simulink model "sim_tcyb_2024_pos_ctrl"  (R2020a)
settings: Solver=ode4  StartTime=0.0  StopTime=30.0  FixedStep=0.01  RelTol=1e-3
values from neighbouring files (symbols this model uses):
  alfa_theta = 20    [init_tcyb_2024_pos_ctrl.m]
  alfa_theta_obs = 100    [init_tcyb_2024_pos_ctrl.m]
  c1_diff_sigma_bar_v = diag([25; 30; 20])    [init_tcyb_2024_pos_ctrl.m]
  c1v = diag([5.8; 6.5; 6.5])    [init_tcyb_2024_pos_ctrl.m]
  c2_diff_sigma_bar_v = diag([50; 50; 10])    [init_tcyb_2024_pos_ctrl.m]
  c2v = diag([5.8; 6.5; 6.5])    [init_tcyb_2024_pos_ctrl.m]
  c3_diff_sigma_bar_v = diag([15; 15; 10])    [init_tcyb_2024_pos_ctrl.m]
  c3v = diag([4.8; 6.4; 6.0])    [init_tcyb_2024_pos_ctrl.m]
  c_psi_p = [0.05; 0.05; 0.05]    [init_tcyb_2024_pos_ctrl.m]
  delta_p_i_0 = zeros(3, NF)    [init_tcyb_2024_pos_ctrl.m]
  delta_v_i_0 = zeros(3, NF)    [init_tcyb_2024_pos_ctrl.m]
  dp_aa_t = 0.2 * ones(3, 5) + ( 1.0 - 0.2 ) * rand(3, 5)    [init_tcyb_2024_pos_ctrl.m]
  dp_ff_t = [ 0.4 * ones(1, 5) + ( 1.0 - 0.4 ) * rand(1, 5);                      0.4 * ones(1, 5) + ( 1.0 - 0.4 ) * rand(1, 5);                      0.2 * ones(1, 5) + ( 0.6 - 0.2 ) * rand(1, 5) ]    [init_tcyb_2024_pos_ctrl.m]
  dp_phi_t = ( - pi / 2 ) * ones(3, 5) + ( pi / 2 - ( - pi / 2 ) ) * rand(3, 5)    [init_tcyb_2024_pos_ctrl.m]
  etai_0 = zeros(3,5)    [init_tcyb_2024_pos_ctrl.m]
  kai_1_t = 0.02    [init_tcyb_2024_pos_ctrl.m]
  kai_3_t = 0.1    [init_tcyb_2024_pos_ctrl.m]
  ksii_0 = zeros(3,5)    [init_tcyb_2024_pos_ctrl.m]
  l1v = diag([20; 20; 20])    [init_tcyb_2024_pos_ctrl.m]
  l2v = diag([30; 30; 30])    [init_tcyb_2024_pos_ctrl.m]
  Lamd_diff_sigma_bar_v = 0.5    [init_tcyb_2024_pos_ctrl.m]
  mass_i = zeros(1,NF)    [init_tcyb_2024_pos_ctrl.m]
  Mii = diag([1;0;0;0;1])    [init_tcyb_2024_pos_ctrl.m]
  pos0 = zeros(3, 1)    [init_tcyb_2024_pos_ctrl.m]
  PZ0 = P0(3)    [init_tcyb_2024_pos_ctrl.m]
  PZ1 = 10    [init_tcyb_2024_pos_ctrl.m]
  Qci_init = repmat([1;0;0;0],1,NF)    [init_tcyb_2024_pos_ctrl.m]
  R0 = 4    [init_tcyb_2024_pos_ctrl.m]
  R1 = 8    [init_tcyb_2024_pos_ctrl.m]
  rho_p = [0.1; 0.1; 0.1]    [init_tcyb_2024_pos_ctrl.m]
  Rx2 = 10    [init_tcyb_2024_pos_ctrl.m]
  Ry2 = 6    [init_tcyb_2024_pos_ctrl.m]
  Rz2 = 4    [init_tcyb_2024_pos_ctrl.m]
  T0 = 0    [init_tcyb_2024_pos_ctrl.m]
  T1 = tseq1    (= 10)    [init_tcyb_2024_pos_ctrl.m]
  T12 = tseq1 + tseq12    (= 20)    [init_tcyb_2024_pos_ctrl.m]
  T2 = tseq1 + tseq12 + tseq2    (= 30)    [init_tcyb_2024_pos_ctrl.m]
  tau_p = 5    [init_tcyb_2024_pos_ctrl.m]
  theta0 = ( 2 / 5 ) * pi    (= 1.25663706144)    [init_tcyb_2024_pos_ctrl.m]
  vel0 = zeros(3, 1)    [init_tcyb_2024_pos_ctrl.m]
  Wij = [0,0,1,0,0;              0,0,1,1,0;              1,0,0,0,1;              0,1,1,0,0;              0,0,1,0,0]    [init_tcyb_2024_pos_ctrl.m]
  X1 = 8    [init_tcyb_2024_pos_ctrl.m]
  X2 = 2    [init_tcyb_2024_pos_ctrl.m]
  X3 = 3    [init_tcyb_2024_pos_ctrl.m]
  Y1 = 10    [init_tcyb_2024_pos_ctrl.m]
  Y2 = 2    [init_tcyb_2024_pos_ctrl.m]
  Y3 = 4    [init_tcyb_2024_pos_ctrl.m]
  Z1 = 4    [init_tcyb_2024_pos_ctrl.m]
  Z2 = -6    [init_tcyb_2024_pos_ctrl.m]
  Z3 = 2    [init_tcyb_2024_pos_ctrl.m]
  zeta_diff_sigma_bar_v = 0.08    [init_tcyb_2024_pos_ctrl.m]
undefined symbols (not defined in the file or in its folder): cal_frac_squ, p_alfav1, p_alfav2, p_gamma1_pos, p_gamma1_vel, p_gamma2_pos, p_gamma2_vel, q_alfav1, q_alfav2, q_gamma1_pos, q_gamma1_vel, q_gamma2_pos, q_gamma2_vel
(part 1 of 4)
settings Model: Creator=zzy  LastModifiedBy=Hershey.A
settings DataIOCC: ReturnWorkspaceOutputs=off
settings DebuggingCC: ArithmeticOperatorsInVariantConditions=warning
settings SFSimCC: SimUseLocalCustomCode=off  CustomCodeUndefinedFunction=UseInterfaceOnly
settings RTWCC: RTWUseLocalCustomCode=off

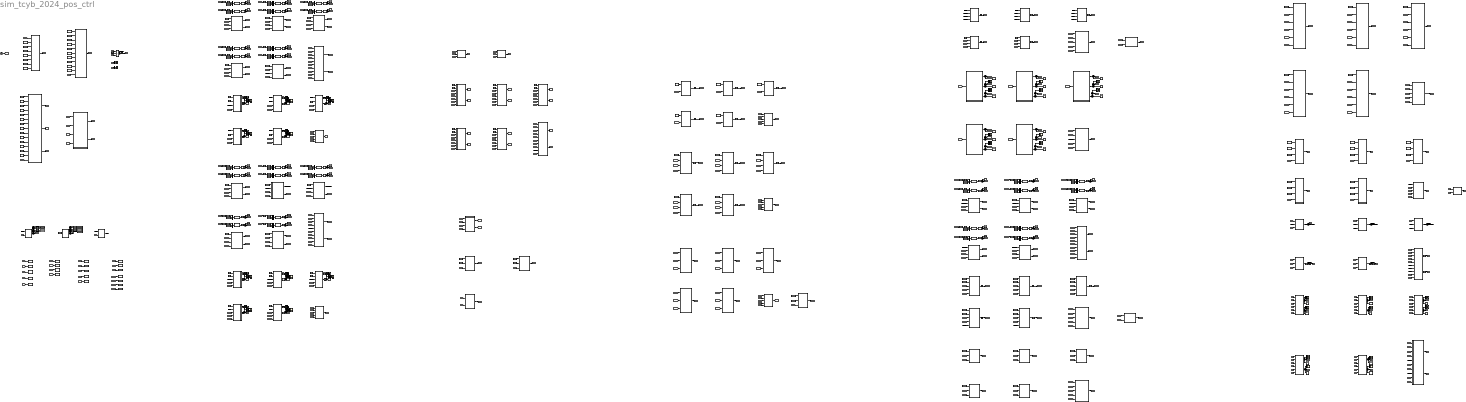
== system sim_tcyb_2024_pos_ctrl ==
  Add{,1..9} (10 alike) : Sum
  Clock : Clock
  Constant : Constant  Value=T1
  Constant{1,4,15,224,228,233,237,242} (8 alike) : Constant  Value=Mii
  Constant{10..14} (5 alike) : Constant  Value=tau_p
  Constant{100,102,107,112,117} (5 alike) : Constant  Value=p_alfav1
  Constant{101,103,108,113,118} (5 alike) : Constant  Value=alfa_theta
  Constant{97,104,109,114,119} (5 alike) : Constant  Value=q_alfav1
  Constant{98,105,110,115,120} (5 alike) : Constant  Value=p_alfav2
  Constant{99,106,111,116,121} (5 alike) : Constant  Value=q_alfav2
  Constant{122,124,126,128,140} (5 alike) : Constant  Value=c1v
  Constant{123,125,127,139,141} (5 alike) : Constant  Value=c2v
  Constant{92..96,142..146} (10 alike) : Constant  Value=c3v
  Constant{2,5,16,223,227,232,236,240} (8 alike) : Constant  Value=Wij
  Constant{17..21} (5 alike) : Constant  Value=c_psi_p
  Constant{182..183,189,199,202,205,209,212,219,252} (10 alike) : Constant  Value=l2v
  Constant{184..186,193..196,198,283..284} (10 alike) : Constant  Value=alfa_theta_obs
  Constant{187,190,197,200,203,206,210,213,230,263} (10 alike) : Constant  Value=l1v
  Constant188 : Constant  Value=delta_p_i_0(:,4)
  Constant191 : Constant  Value=mass_i
  Constant192 : Constant  Value=delta_p_i_0(:,5)
  Constant201 : Constant  Value=delta_v_i_0(:,1)
  Constant204 : Constant  Value=delta_v_i_0(:,2)
  Constant207 : Constant  Value=delta_v_i_0(:,3)
  Constant208 : Constant  Value=delta_p_i_0(:,1)
  Constant211 : Constant  Value=delta_v_i_0(:,4)
  Constant214 : Constant  Value=delta_v_i_0(:,5)
  Constant{215,220,270,275,279} (5 alike) : Constant  Value=p_gamma1_pos
  Constant{216,267,271,276,280} (5 alike) : Constant  Value=q_gamma1_pos
  Constant{217,268,272,277,281} (5 alike) : Constant  Value=p_gamma2_pos
  Constant{218,269,273,278,282} (5 alike) : Constant  Value=q_gamma2_pos
  Constant221 : Constant  Value=Z1
  Constant222 : Constant  Value=Z2
  Constant225 : Constant  Value=theta0
  Constant226 : Constant  Value=Z3
  Constant229 : Constant  Value=Y3
  Constant231 : Constant  Value=kai_1_t
  Constant234 : Constant  Value=X3
  Constant235 : Constant  Value=kai_3_t
  Constant238 : Constant  Value=T1
  Constant239 : Constant  Value=T12
  Constant24 : Constant  Value=R0
  Constant241 : Constant  Value=delta_p_i_0(:,2)
  Constant{243,286,289,292,295} (5 alike) : Constant  Value=dp_phi_t
  Constant{244,287,290,293,296} (5 alike) : Constant  Value=dp_ff_t
  Constant{245,249,254,258,262} (5 alike) : Constant  Value=p_gamma1_vel
  Constant{246,250,255,259,264} (5 alike) : Constant  Value=q_gamma1_vel
  Constant{247,251,256,260,265} (5 alike) : Constant  Value=p_gamma2_vel
  Constant{248,253,257,261,266} (5 alike) : Constant  Value=q_gamma2_vel
  Constant25 : Constant  Value=R1
  Constant26 : Constant  Value=T0
  Constant27 : Constant  Value=Rz2
  Constant274 : Constant  Value=delta_p_i_0(:,3)
  Constant28 : Constant  Value=Ry2
  Constant{285,288,291,294,297} (5 alike) : Constant  Value=dp_aa_t
  Constant29 : Constant  Value=Rx2
  Constant{3,6..9} (5 alike) : Constant  Value=rho_p
  Constant30 : Constant  Value=X1
  Constant31 : Constant  Value=X2
  Constant32 : Constant  Value=Y1
  Constant33 : Constant  Value=Y2
  Constant51 : Constant  Value=Qci_init
  Constant64 : Constant  Value=T2
  Constant65 : Constant  Value=R0
  Constant66 : Constant  Value=R1
  Constant67 : Constant  Value=Rx2
  Constant68 : Constant  Value=Ry2
  Constant69 : Constant  Value=Rz2
  Constant70 : Constant  Value=T2
  Constant71 : Constant  Value=T1
  Constant72 : Constant  Value=PZ0
  Constant73 : Constant  Value=PZ1
  Demux{1..10,12,22..32,68..80,88,92..97} (42 alike) : Demux  Outputs=3
  Display{6,12..25,35..59,64..68,76..95} (65 alike) : Display
  Interpreted MATLAB Function{20..29,41..60} (30 alike) : MATLABFcn  MATLABFcn=cal_frac_squ(u(1:3),u(4),u(5))
  Memory1 : Memory  InitialCondition=etai_0
  Memory2 : Memory  InitialCondition=ksii_0
  Mux{86..108,119,130..135} (30 alike) : Mux  Inputs=2
  Mux{19..28,109..118,120..129} (30 alike) : Mux  Inputs=3
  Step : Step  Time=T1+0.01  SampleTime=0
  To Workspace : ToWorkspace  VariableName=eta_d_est_vec  SampleTime=-1
  To Workspace1 : ToWorkspace  VariableName=dp_hat_vec  SampleTime=-1
  To Workspace10 : ToWorkspace  VariableName=eta_track_err_vec  SampleTime=-1
  To Workspace11 : ToWorkspace  VariableName=sigma_bar_v_hat_vec  SampleTime=-1
  To Workspace12 : ToWorkspace  VariableName=sigma_bar_v_vec  SampleTime=-1
  To Workspace13 : ToWorkspace  VariableName=sigma_bar_v_tilt_vec  SampleTime=-1
  To Workspace14 : ToWorkspace  VariableName=ui_vec  SampleTime=-1
  To Workspace17 : ToWorkspace  VariableName=ksi_est_err  SampleTime=-1
  To Workspace18 : ToWorkspace  VariableName=ksi_d_est_vec  SampleTime=-1
  To Workspace19 : ToWorkspace  VariableName=sigma_v_vec  SampleTime=-1
  To Workspace2 : ToWorkspace  VariableName=dp_vec  SampleTime=-1
  To Workspace20 : ToWorkspace  VariableName=delta_ksi_vec  SampleTime=-1
  To Workspace21 : ToWorkspace  VariableName=delta_eta_vec  SampleTime=-1
  To Workspace22 : ToWorkspace  VariableName=eta_est_err  SampleTime=-1
  To Workspace3 : ToWorkspace  VariableName=u0  SampleTime=-1
  To Workspace4 : ToWorkspace  VariableName=eta0  SampleTime=-1
  To Workspace5 : ToWorkspace  VariableName=ksi0  SampleTime=-1
  To Workspace6 : ToWorkspace  VariableName=dp_tilt_vec  SampleTime=-1
  To Workspace7 : ToWorkspace  VariableName=eta_i_vec  SampleTime=-1
  To Workspace8 : ToWorkspace  VariableName=ksi_i_vec  SampleTime=-1
  To Workspace9 : ToWorkspace  VariableName=ksi_track_err_vec  SampleTime=-1
  cal Rci from ui : MATLAB Function  TreatAsAtomicUnit=on
  cal Rei : MATLAB Function  TreatAsAtomicUnit=on
  cal Ri : MATLAB Function  TreatAsAtomicUnit=on
  cal abs 21 : MATLAB Function  TreatAsAtomicUnit=on
  cal abs 22 : MATLAB Function  TreatAsAtomicUnit=on
  cal abs 23 : MATLAB Function  TreatAsAtomicUnit=on
  cal abs 24 : MATLAB Function  TreatAsAtomicUnit=on
  cal abs 25 : MATLAB Function  TreatAsAtomicUnit=on
  cal abs 26 : MATLAB Function  TreatAsAtomicUnit=on
  cal abs 27 : MATLAB Function  TreatAsAtomicUnit=on
  cal abs 28 : MATLAB Function  TreatAsAtomicUnit=on
  cal abs 29 : MATLAB Function  TreatAsAtomicUnit=on
  cal abs 30 : MATLAB Function  TreatAsAtomicUnit=on
  cal abs 41 : MATLAB Function  TreatAsAtomicUnit=on
  cal abs 42 : MATLAB Function  TreatAsAtomicUnit=on
  cal abs 43 : MATLAB Function  TreatAsAtomicUnit=on
  cal abs 44 : MATLAB Function  TreatAsAtomicUnit=on
  cal abs 45 : MATLAB Function  TreatAsAtomicUnit=on
  cal abs 46 : MATLAB Function  TreatAsAtomicUnit=on
  cal abs 47 : MATLAB Function  TreatAsAtomicUnit=on
  cal abs 48 : MATLAB Function  TreatAsAtomicUnit=on
  cal abs 49 : MATLAB Function  TreatAsAtomicUnit=on
  cal abs 50 : MATLAB Function  TreatAsAtomicUnit=on
  cal abs 51 : MATLAB Function  TreatAsAtomicUnit=on
  cal abs 52 : MATLAB Function  TreatAsAtomicUnit=on
  cal abs 53 : MATLAB Function  TreatAsAtomicUnit=on
  cal abs 54 : MATLAB Function  TreatAsAtomicUnit=on
  cal abs 55 : MATLAB Function  TreatAsAtomicUnit=on
  cal abs 56 : MATLAB Function  TreatAsAtomicUnit=on
  cal abs 57 : MATLAB Function  TreatAsAtomicUnit=on
  cal abs 58 : MATLAB Function  TreatAsAtomicUnit=on
  cal abs 59 : MATLAB Function  TreatAsAtomicUnit=on
  cal abs 60 : MATLAB Function  TreatAsAtomicUnit=on
  cal auxiliary error Gi agent 1 : MATLAB Function  TreatAsAtomicUnit=on
  cal auxiliary error Gi agent 2 : MATLAB Function  TreatAsAtomicUnit=on
  cal auxiliary error Gi agent 3 : MATLAB Function  TreatAsAtomicUnit=on
  cal auxiliary error Gi agent 4 : MATLAB Function  TreatAsAtomicUnit=on
  cal auxiliary error Gi agent 5 : MATLAB Function  TreatAsAtomicUnit=on
  cal combine sigma_bar_v : MATLAB Function  TreatAsAtomicUnit=on
  cal combine sigma_bar_v_tilt : MATLAB Function  TreatAsAtomicUnit=on
  cal differentiator d_sigma_bar_v_hat agent 1 : Subsystem
  cal differentiator d_sigma_bar_v_hat agent 2 : Subsystem
  cal differentiator d_sigma_bar_v_hat agent 3 : Subsystem
  cal differentiator d_sigma_bar_v_hat agent 4 : Subsystem
  cal differentiator d_sigma_bar_v_hat agent 5 : Subsystem
  cal disturbance observation error dp_tilt : MATLAB Function  TreatAsAtomicUnit=on
  cal dp_hat agent 1 : MATLAB Function  TreatAsAtomicUnit=on
  cal dp_hat agent 2 : MATLAB Function  TreatAsAtomicUnit=on
  cal dp_hat agent 3 : MATLAB Function  TreatAsAtomicUnit=on
  cal dp_hat agent 4 : MATLAB Function  TreatAsAtomicUnit=on
  cal dp_hat agent 5 : MATLAB Function  TreatAsAtomicUnit=on
  cal formation tracking Gi error : MATLAB Function  TreatAsAtomicUnit=on
  cal formation tracking position errors : MATLAB Function  TreatAsAtomicUnit=on
  cal formation tracking velocity errors : MATLAB Function  TreatAsAtomicUnit=on
  cal lump formation error : MATLAB Function  TreatAsAtomicUnit=on
  cal lumped observation error agent 1 : MATLAB Function  TreatAsAtomicUnit=on
  cal lumped observation error agent 2 : MATLAB Function  TreatAsAtomicUnit=on
  cal lumped observation error agent 3 : MATLAB Function  TreatAsAtomicUnit=on
  cal lumped observation error agent 4 : MATLAB Function  TreatAsAtomicUnit=on
  cal lumped observation error agent 5 : MATLAB Function  TreatAsAtomicUnit=on
  cal position and velocity signal tracking errors : MATLAB Function  TreatAsAtomicUnit=on
  cal position estimate error : MATLAB Function  TreatAsAtomicUnit=on
  cal sigma_bar_v_hat agent 1 : MATLAB Function  TreatAsAtomicUnit=on
  cal sigma_bar_v_hat agent 2 : MATLAB Function  TreatAsAtomicUnit=on
  cal sigma_bar_v_hat agent 3 : MATLAB Function  TreatAsAtomicUnit=on
  cal sigma_bar_v_hat agent 4 : MATLAB Function  TreatAsAtomicUnit=on
  cal sigma_bar_v_hat agent 5 : MATLAB Function  TreatAsAtomicUnit=on
  cal theta_eta_est_err_tilt agent 1 : MATLAB Function  TreatAsAtomicUnit=on
  cal theta_eta_est_err_tilt agent 2 : MATLAB Function  TreatAsAtomicUnit=on
  cal theta_eta_est_err_tilt agent 3 : MATLAB Function  TreatAsAtomicUnit=on
  cal theta_eta_est_err_tilt agent 4 : MATLAB Function  TreatAsAtomicUnit=on
  cal theta_eta_est_err_tilt agent 5 : MATLAB Function  TreatAsAtomicUnit=on
  cal theta_ksi_est_err_tilt agent 1 : MATLAB Function  TreatAsAtomicUnit=on
  cal theta_ksi_est_err_tilt agent 2 : MATLAB Function  TreatAsAtomicUnit=on
  cal theta_ksi_est_err_tilt agent 3 : MATLAB Function  TreatAsAtomicUnit=on
  cal theta_ksi_est_err_tilt agent 4 : MATLAB Function  TreatAsAtomicUnit=on
  cal theta_ksi_est_err_tilt agent 5 : MATLAB Function  TreatAsAtomicUnit=on
  cal theta_sigma_bar_v_tilt agent 1 : MATLAB Function  TreatAsAtomicUnit=on
  cal theta_sigma_bar_v_tilt agent 2 : MATLAB Function  TreatAsAtomicUnit=on
  cal theta_sigma_bar_v_tilt agent 3 : MATLAB Function  TreatAsAtomicUnit=on
  cal theta_sigma_bar_v_tilt agent 4 : MATLAB Function  TreatAsAtomicUnit=on
  cal theta_sigma_bar_v_tilt agent 5 : MATLAB Function  TreatAsAtomicUnit=on
  cal ui agent 1 : MATLAB Function  TreatAsAtomicUnit=on
  cal ui agent 2 : MATLAB Function  TreatAsAtomicUnit=on
  cal ui agent 3 : MATLAB Function  TreatAsAtomicUnit=on
  cal ui agent 4 : MATLAB Function  TreatAsAtomicUnit=on
  cal ui agent 5 : MATLAB Function  TreatAsAtomicUnit=on
  cal velocity estimate error : MATLAB Function  TreatAsAtomicUnit=on
  cal virtual control sigma_v agent 1 : MATLAB Function  TreatAsAtomicUnit=on
  cal virtual control sigma_v agent 2 : MATLAB Function  TreatAsAtomicUnit=on
  cal virtual control sigma_v agent 3 : MATLAB Function  TreatAsAtomicUnit=on
  cal virtual control sigma_v agent 4 : MATLAB Function  TreatAsAtomicUnit=on
  cal virtual control sigma_v agent 5 : MATLAB Function  TreatAsAtomicUnit=on
  choose eta_est_err_tilt 1 : MATLAB Function  TreatAsAtomicUnit=on
  choose eta_est_err_tilt 10 : MATLAB Function  TreatAsAtomicUnit=on
  choose eta_est_err_tilt 11 : MATLAB Function  TreatAsAtomicUnit=on
  choose eta_est_err_tilt 12 : MATLAB Function  TreatAsAtomicUnit=on
  choose eta_est_err_tilt 13 : MATLAB Function  TreatAsAtomicUnit=on
  choose eta_est_err_tilt 14 : MATLAB Function  TreatAsAtomicUnit=on
  choose eta_est_err_tilt 15 : MATLAB Function  TreatAsAtomicUnit=on
  choose eta_est_err_tilt 16 : MATLAB Function  TreatAsAtomicUnit=on
  choose eta_est_err_tilt 17 : MATLAB Function  TreatAsAtomicUnit=on
  choose eta_est_err_tilt 18 : MATLAB Function  TreatAsAtomicUnit=on
  choose eta_est_err_tilt 19 : MATLAB Function  TreatAsAtomicUnit=on
  choose eta_est_err_tilt 2 : MATLAB Function  TreatAsAtomicUnit=on
  choose eta_est_err_tilt 20 : MATLAB Function  TreatAsAtomicUnit=on
  choose eta_est_err_tilt 3 : MATLAB Function  TreatAsAtomicUnit=on
  choose eta_est_err_tilt 4 : MATLAB Function  TreatAsAtomicUnit=on
  choose eta_est_err_tilt 5 : MATLAB Function  TreatAsAtomicUnit=on
  choose eta_est_err_tilt 6 : MATLAB Function  TreatAsAtomicUnit=on
  choose eta_est_err_tilt 7 : MATLAB Function  TreatAsAtomicUnit=on
  choose eta_est_err_tilt 8 : MATLAB Function  TreatAsAtomicUnit=on
  choose eta_est_err_tilt 9 : MATLAB Function  TreatAsAtomicUnit=on
  choose ksi_est_err 21 : MATLAB Function  TreatAsAtomicUnit=on
  choose ksi_est_err 22 : MATLAB Function  TreatAsAtomicUnit=on
  choose ksi_est_err 23 : MATLAB Function  TreatAsAtomicUnit=on
  choose ksi_est_err 24 : MATLAB Function  TreatAsAtomicUnit=on
  choose ksi_est_err 25 : MATLAB Function  TreatAsAtomicUnit=on
  choose ksi_est_err 26 : MATLAB Function  TreatAsAtomicUnit=on
  choose ksi_est_err 27 : MATLAB Function  TreatAsAtomicUnit=on
  choose ksi_est_err 28 : MATLAB Function  TreatAsAtomicUnit=on
  choose ksi_est_err 29 : MATLAB Function  TreatAsAtomicUnit=on
  choose ksi_est_err 30 : MATLAB Function  TreatAsAtomicUnit=on
  combine Gi : MATLAB Function  TreatAsAtomicUnit=on
  combine d_sigma_bar_v_est : MATLAB Function  TreatAsAtomicUnit=on
  combine dp_hat : MATLAB Function  TreatAsAtomicUnit=on
  combine eps_p_hat adaptive : MATLAB Function  TreatAsAtomicUnit=on
  combine eta_p_hat adaptive : MATLAB Function  TreatAsAtomicUnit=on
  combine follower desire velocity estimaters : MATLAB Function  TreatAsAtomicUnit=on
  combine follower eta ksi : MATLAB Function  TreatAsAtomicUnit=on
  combine formation control input : MATLAB Function  TreatAsAtomicUnit=on
  combine leader position estimaters : MATLAB Function  TreatAsAtomicUnit=on
  "combine lumped follower observation error " : MATLAB Function  TreatAsAtomicUnit=on
  combine lumped follower position observation error : MATLAB Function  TreatAsAtomicUnit=on
  combine lumped follower velocity observation error : MATLAB Function  TreatAsAtomicUnit=on
  combine sigma_bar_v_hat : MATLAB Function  TreatAsAtomicUnit=on
  combine sigma_v : MATLAB Function  TreatAsAtomicUnit=on
  combine theta_sigma_bar_v_tilt : MATLAB Function  TreatAsAtomicUnit=on
  combine translational disturbance : MATLAB Function  TreatAsAtomicUnit=on
  combine ui : MATLAB Function  TreatAsAtomicUnit=on
  d2_sigma_bar_v_est_{1..5} (5 alike) : Scope  NumInputPorts=3
  d_sigma_bar_v_est_{1..5} (5 alike) : Scope  NumInputPorts=3
  depart Rc1 : MATLAB Function  TreatAsAtomicUnit=on
  depart Rc2 : MATLAB Function  TreatAsAtomicUnit=on
  depart Rc3 : MATLAB Function  TreatAsAtomicUnit=on
  depart Rc4 : MATLAB Function  TreatAsAtomicUnit=on
  depart Rc5 : MATLAB Function  TreatAsAtomicUnit=on
  depart Re1 : MATLAB Function  TreatAsAtomicUnit=on
  depart Re2 : MATLAB Function  TreatAsAtomicUnit=on
  depart Re3 : MATLAB Function  TreatAsAtomicUnit=on
  depart Re4 : MATLAB Function  TreatAsAtomicUnit=on
  depart Re5 : MATLAB Function  TreatAsAtomicUnit=on
  desire formation position and velocity : MATLAB Function  TreatAsAtomicUnit=on
  eps_p_hat Integrator{,1..4} (5 alike) : Integrator  InitialCondition=zeros(3,1)
  eps_p_hat adaptive law agent 1 : MATLAB Function  TreatAsAtomicUnit=on
  eps_p_hat adaptive law agent 2 : MATLAB Function  TreatAsAtomicUnit=on
  eps_p_hat adaptive law agent 3 : MATLAB Function  TreatAsAtomicUnit=on
  eps_p_hat adaptive law agent 4 : MATLAB Function  TreatAsAtomicUnit=on
  eps_p_hat adaptive law agent 5 : MATLAB Function  TreatAsAtomicUnit=on
  eta_0 : Scope  NumInputPorts=3
  eta_d_est_{1..5} (5 alike) : Scope  NumInputPorts=3
  eta_p_hat Integrator{,1..4} (5 alike) : Integrator  InitialCondition=zeros(3,1)
  eta_p_hat adaptive law agent 1 : MATLAB Function  TreatAsAtomicUnit=on
  eta_p_hat adaptive law agent 2 : MATLAB Function  TreatAsAtomicUnit=on
  eta_p_hat adaptive law agent 3 : MATLAB Function  TreatAsAtomicUnit=on
  eta_p_hat adaptive law agent 4 : MATLAB Function  TreatAsAtomicUnit=on
  eta_p_hat adaptive law agent 5 : MATLAB Function  TreatAsAtomicUnit=on
  eta_track_err_{1..5} (5 alike) : Scope  NumInputPorts=3
  fixed-time distributed follower desire position observer agent 1 : MATLAB Function  TreatAsAtomicUnit=on
  fixed-time distributed follower desire position observer agent 2 : MATLAB Function  TreatAsAtomicUnit=on
  fixed-time distributed follower desire position observer agent 3 : MATLAB Function  TreatAsAtomicUnit=on
  fixed-time distributed follower desire position observer agent 4 : MATLAB Function  TreatAsAtomicUnit=on
  fixed-time distributed follower desire position observer agent 5 : MATLAB Function  TreatAsAtomicUnit=on
  fixed-time distributed follower desire velocity observer agent 1 : MATLAB Function  TreatAsAtomicUnit=on
  fixed-time distributed follower desire velocity observer agent 2 : MATLAB Function  TreatAsAtomicUnit=on
  fixed-time distributed follower desire velocity observer agent 3 : MATLAB Function  TreatAsAtomicUnit=on
  fixed-time distributed follower desire velocity observer agent 4 : MATLAB Function  TreatAsAtomicUnit=on
  fixed-time distributed follower desire velocity observer agent 5 : MATLAB Function  TreatAsAtomicUnit=on
  follower etai Integrator agent 1 : Integrator  InitialCondition=etai_0(:,1)
  follower etai Integrator agent 2 : Integrator  InitialCondition=etai_0(:,2)
  follower etai Integrator agent 3 : Integrator  InitialCondition=etai_0(:,3)
  follower etai Integrator agent 4 : Integrator  InitialCondition=etai_0(:,4)
  follower etai Integrator agent 5 : Integrator  InitialCondition=etai_0(:,5)
  follower ksii Integrator agent 1 : Integrator  InitialCondition=ksii_0(:,1)
  follower ksii Integrator agent 2 : Integrator  InitialCondition=ksii_0(:,2)
  follower ksii Integrator agent 3 : Integrator  InitialCondition=ksii_0(:,3)
  follower ksii Integrator agent 4 : Integrator  InitialCondition=ksii_0(:,4)
  follower ksii Integrator agent 5 : Integrator  InitialCondition=ksii_0(:,5)
  follower tracking error agent 1 : MATLAB Function  TreatAsAtomicUnit=on
  follower tracking error agent 2 : MATLAB Function  TreatAsAtomicUnit=on
  follower tracking error agent 3 : MATLAB Function  TreatAsAtomicUnit=on
  follower tracking error agent 4 : MATLAB Function  TreatAsAtomicUnit=on
  follower tracking error agent 5 : MATLAB Function  TreatAsAtomicUnit=on
  generate translational disturbance agent 1 : MATLAB Function  TreatAsAtomicUnit=on
  generate translational disturbance agent 2 : MATLAB Function  TreatAsAtomicUnit=on
  generate translational disturbance agent 3 : MATLAB Function  TreatAsAtomicUnit=on
  generate translational disturbance agent 4 : MATLAB Function  TreatAsAtomicUnit=on
  generate translational disturbance agent 5 : MATLAB Function  TreatAsAtomicUnit=on
  ksi_0 : Scope  NumInputPorts=3
  ksi_d_est_{1..5} (5 alike) : Scope  NumInputPorts=3
  ksi_track_err_{1..5} (5 alike) : Scope  NumInputPorts=3
  leader control input : MATLAB Function  TreatAsAtomicUnit=on
  leader eta0 Integrator : Integrator  ExternalReset=rising  InitialConditionSource=external  InitialCondition=vel0
  leader ksi0 Integrator : Integrator  InitialCondition=pos0
  position observe Integrator {1..5} (5 alike) : Integrator  InitialCondition=zeros(3,1)
  process velocity : MATLAB Function  TreatAsAtomicUnit=on
  set desire formation configuration : MATLAB Function  TreatAsAtomicUnit=on
  sigma_bar_v_hat Integrator {1..5} (5 alike) : Integrator  InitialCondition=zeros(3,1)
  sigma_v Integrator {1..5} (5 alike) : Integrator  InitialCondition=zeros(3,1)
  trans to column20 : MATLAB Function  TreatAsAtomicUnit=on
  trans to column21 : MATLAB Function  TreatAsAtomicUnit=on
  trans to column22 : MATLAB Function  TreatAsAtomicUnit=on
  trans to column23 : MATLAB Function  TreatAsAtomicUnit=on
  trans to column24 : MATLAB Function  TreatAsAtomicUnit=on
  trans to column25 : MATLAB Function  TreatAsAtomicUnit=on
  trans to column26 : MATLAB Function  TreatAsAtomicUnit=on
  trans to column27 : MATLAB Function  TreatAsAtomicUnit=on
  trans to column28 : MATLAB Function  TreatAsAtomicUnit=on
  trans to column29 : MATLAB Function  TreatAsAtomicUnit=on
  trans to column41 : MATLAB Function  TreatAsAtomicUnit=on
  trans to column42 : MATLAB Function  TreatAsAtomicUnit=on
  trans to column43 : MATLAB Function  TreatAsAtomicUnit=on
  trans to column44 : MATLAB Function  TreatAsAtomicUnit=on
  trans to column45 : MATLAB Function  TreatAsAtomicUnit=on
  trans to column46 : MATLAB Function  TreatAsAtomicUnit=on
  trans to column47 : MATLAB Function  TreatAsAtomicUnit=on
  trans to column48 : MATLAB Function  TreatAsAtomicUnit=on
  trans to column49 : MATLAB Function  TreatAsAtomicUnit=on
  trans to column50 : MATLAB Function  TreatAsAtomicUnit=on
  trans to column51 : MATLAB Function  TreatAsAtomicUnit=on
  trans to column52 : MATLAB Function  TreatAsAtomicUnit=on
  trans to column53 : MATLAB Function  TreatAsAtomicUnit=on
  trans to column54 : MATLAB Function  TreatAsAtomicUnit=on
  trans to column55 : MATLAB Function  TreatAsAtomicUnit=on
  trans to column56 : MATLAB Function  TreatAsAtomicUnit=on
  trans to column57 : MATLAB Function  TreatAsAtomicUnit=on
  trans to column58 : MATLAB Function  TreatAsAtomicUnit=on
  trans to column59 : MATLAB Function  TreatAsAtomicUnit=on
  trans to column60 : MATLAB Function  TreatAsAtomicUnit=on
  uav translational dynamics agent 1 : MATLAB Function  TreatAsAtomicUnit=on
  uav translational dynamics agent 2 : MATLAB Function  TreatAsAtomicUnit=on
  uav translational dynamics agent 3 : MATLAB Function  TreatAsAtomicUnit=on
  uav translational dynamics agent 4 : MATLAB Function  TreatAsAtomicUnit=on
  uav translational dynamics agent 5 : MATLAB Function  TreatAsAtomicUnit=on
  velocity observe Integrator {1..5} (5 alike) : Integrator  InitialCondition=zeros(3,1)
  wires:
  cal ui agent 1/1(ui_1) -> [ui_1]
  [ui_5] -> combine ui/5(ui_5)
  [ui_2] -> combine ui/2(ui_2)
  [ui_1] -> combine ui/1(ui_1)
  [ui_4] -> combine ui/4(ui_4)
  [ui_3] -> combine ui/3(ui_3)
  [eta_i_vec] -> cal position and velocity signal tracking errors/3(eta_i_vec)
  [ksi_i_vec] -> cal position and velocity signal tracking errors/1(ksi_i_vec)
  [ksi_d_est_vec] -> cal position and velocity signal tracking errors/2(ksi_d_est_vec)
  [eta_d_est_vec] -> cal position and velocity signal tracking errors/4(eta_d_est_vec)
  Constant4/1 -> cal formation tracking position errors/1(wi0)
  Constant5/1 -> cal formation tracking position errors/2(wij)
  cal position and velocity signal tracking errors/1(err_ksi_vec) -> [err_ksi_vec]
  [err_ksi_vec] -> cal formation tracking position errors/3(err_ksi_vec)
  cal formation tracking position errors/1(err_ksi_form_vec) -> [err_ksi_form_vec]
  cal position and velocity signal tracking errors/2(err_eta_vec) -> [err_eta_vec]
  cal formation tracking velocity errors/1(err_eta_form_vec) -> [err_eta_form_vec]
  [err_eta_vec] -> cal formation tracking velocity errors/3(err_eta_vec)
  Constant2/1 -> cal formation tracking velocity errors/2(wij)
  Constant1/1 -> cal formation tracking velocity errors/1(wi0)
  [err_ksi_form_vec] -> cal lump formation error/1(err_ksi_form_vec)
  [err_eta_form_vec] -> cal lump formation error/2(err_eta_form_vec)
  cal lump formation error/1(err_lump_vec) -> [err_lump_vec]
  [err_lump_vec] -> eps_p_hat adaptive law agent 1/2(err_lump_vec)
  Constant3/1 -> eps_p_hat adaptive law agent 1/1(rho_p)
  eps_p_hat adaptive law agent 1/1(d_eps_p_hat_1) -> eps_p_hat Integrator/1
  eps_p_hat adaptive law agent 2/1(d_eps_p_hat_2) -> eps_p_hat Integrator1/1
  [err_lump_vec] -> eps_p_hat adaptive law agent 2/2(err_lump_vec)
  Constant6/1 -> eps_p_hat adaptive law agent 2/1(rho_p)
  Constant7/1 -> eps_p_hat adaptive law agent 3/1(rho_p)
  [err_lump_vec] -> eps_p_hat adaptive law agent 3/2(err_lump_vec)
  eps_p_hat adaptive law agent 3/1(d_eps_p_hat_3) -> eps_p_hat Integrator2/1
  eps_p_hat adaptive law agent 4/1(d_eps_p_hat_4) -> eps_p_hat Integrator3/1
  Constant8/1 -> eps_p_hat adaptive law agent 4/1(rho_p)
  [err_lump_vec] -> eps_p_hat adaptive law agent 4/2(err_lump_vec)
  Constant9/1 -> eps_p_hat adaptive law agent 5/1(rho_p)
  [err_lump_vec] -> eps_p_hat adaptive law agent 5/2(err_lump_vec)
  eps_p_hat adaptive law agent 5/1(d_eps_p_hat_5) -> eps_p_hat Integrator4/1
  [eps_p_hat_3] -> combine eps_p_hat adaptive/3(eps_p_hat_3)
  [eps_p_hat_1] -> combine eps_p_hat adaptive/1(eps_p_hat_1)
  [eps_p_hat_5] -> combine eps_p_hat adaptive/5(eps_p_hat_5)
  [eps_p_hat_4] -> combine eps_p_hat adaptive/4(eps_p_hat_4)
  combine eps_p_hat adaptive/1(eps_p_hat_vec) -> [eps_p_hat_vec]
  [eps_p_hat_2] -> combine eps_p_hat adaptive/2(eps_p_hat_2)
  eps_p_hat Integrator/1 -> [eps_p_hat_1]
  eps_p_hat Integrator1/1 -> [eps_p_hat_2]
  eps_p_hat Integrator2/1 -> [eps_p_hat_3]
  eps_p_hat Integrator3/1 -> [eps_p_hat_4]
  eps_p_hat Integrator4/1 -> [eps_p_hat_5]
  Constant10/1 -> eta_p_hat adaptive law agent 1/1(tau_p)
  [tsim] -> eta_p_hat adaptive law agent 1/2(tsim)
  [err_lump_vec] -> eta_p_hat adaptive law agent 1/3(err_lump_vec)
  [eta_p_hat_vec] -> eta_p_hat adaptive law agent 1/4(eta_p_hat_vec)
  eta_p_hat adaptive law agent 1/1(d_eta_p_hat_1) -> eta_p_hat Integrator/1
  eta_p_hat Integrator/1 -> [eta_p_hat_1]
  [err_lump_vec] -> eta_p_hat adaptive law agent 2/3(err_lump_vec)
  Constant11/1 -> eta_p_hat adaptive law agent 2/1(tau_p)
  [eta_p_hat_vec] -> eta_p_hat adaptive law agent 2/4(eta_p_hat_vec)
  eta_p_hat Integrator1/1 -> [eta_p_hat_2]
  eta_p_hat adaptive law agent 2/1(d_eta_p_hat_2) -> eta_p_hat Integrator1/1
  [tsim] -> eta_p_hat adaptive law agent 2/2(tsim)
  eta_p_hat adaptive law agent 3/1(d_eta_p_hat_3) -> eta_p_hat Integrator2/1
  [tsim] -> eta_p_hat adaptive law agent 3/2(tsim)
  eta_p_hat Integrator2/1 -> [eta_p_hat_3]
  [err_lump_vec] -> eta_p_hat adaptive law agent 3/3(err_lump_vec)
  Constant12/1 -> eta_p_hat adaptive law agent 3/1(tau_p)
  [eta_p_hat_vec] -> eta_p_hat adaptive law agent 3/4(eta_p_hat_vec)
  eta_p_hat Integrator3/1 -> [eta_p_hat_4]
  eta_p_hat adaptive law agent 4/1(d_eta_p_hat_4) -> eta_p_hat Integrator3/1
  [eta_p_hat_vec] -> eta_p_hat adaptive law agent 4/4(eta_p_hat_vec)
  Constant13/1 -> eta_p_hat adaptive law agent 4/1(tau_p)
  [err_lump_vec] -> eta_p_hat adaptive law agent 4/3(err_lump_vec)
  [tsim] -> eta_p_hat adaptive law agent 4/2(tsim)
  eta_p_hat Integrator4/1 -> [eta_p_hat_5]
  eta_p_hat adaptive law agent 5/1(d_eta_p_hat_5) -> eta_p_hat Integrator4/1
  [tsim] -> eta_p_hat adaptive law agent 5/2(tsim)
  [eta_p_hat_vec] -> eta_p_hat adaptive law agent 5/4(eta_p_hat_vec)
  Constant14/1 -> eta_p_hat adaptive law agent 5/1(tau_p)
  [err_lump_vec] -> eta_p_hat adaptive law agent 5/3(err_lump_vec)
  [eta_p_hat_2] -> combine eta_p_hat adaptive/2(eta_p_hat_2)
  [eta_p_hat_4] -> combine eta_p_hat adaptive/4(eta_p_hat_4)
  [eta_p_hat_1] -> combine eta_p_hat adaptive/1(eta_p_hat_1)
  [eta_p_hat_5] -> combine eta_p_hat adaptive/5(eta_p_hat_5)
  combine eta_p_hat adaptive/1(eta_p_hat_vec) -> [eta_p_hat_vec]
  [eta_p_hat_3] -> combine eta_p_hat adaptive/3(eta_p_hat_3)
  cal auxiliary error Gi agent 1/1(Gi_1) -> [Gi_1]
  [tsim] -> cal auxiliary error Gi agent 1/1(tsim)
  [err_lump_vec] -> cal auxiliary error Gi agent 1/2(err_lump_vec)
  [eta_p_hat_vec] -> cal auxiliary error Gi agent 1/3(eta_p_hat_vec)
  [tsim] -> cal auxiliary error Gi agent 2/1(tsim)
  [err_lump_vec] -> cal auxiliary error Gi agent 2/2(err_lump_vec)
  cal auxiliary error Gi agent 2/1(Gi_2) -> [Gi_2]
  [eta_p_hat_vec] -> cal auxiliary error Gi agent 2/3(eta_p_hat_vec)
  cal auxiliary error Gi agent 3/1(Gi_3) -> [Gi_3]
  [eta_p_hat_vec] -> cal auxiliary error Gi agent 3/3(eta_p_hat_vec)
  [err_lump_vec] -> cal auxiliary error Gi agent 3/2(err_lump_vec)
  [tsim] -> cal auxiliary error Gi agent 3/1(tsim)
  [eta_p_hat_vec] -> cal auxiliary error Gi agent 4/3(eta_p_hat_vec)
  [tsim] -> cal auxiliary error Gi agent 4/1(tsim)
  cal auxiliary error Gi agent 4/1(Gi_4) -> [Gi_4]
  [err_lump_vec] -> cal auxiliary error Gi agent 4/2(err_lump_vec)
  cal auxiliary error Gi agent 5/1(Gi_5) -> [Gi_5]
  [eta_p_hat_vec] -> cal auxiliary error Gi agent 5/3(eta_p_hat_vec)
  [err_lump_vec] -> cal auxiliary error Gi agent 5/2(err_lump_vec)
  [tsim] -> cal auxiliary error Gi agent 5/1(tsim)
  [Gi_5] -> combine Gi/5(Gi_5)
  [Gi_3] -> combine Gi/3(Gi_3)
  combine Gi/1(Gi_vec) -> [Gi_vec]
  [Gi_2] -> combine Gi/2(Gi_2)
  [Gi_4] -> combine Gi/4(Gi_4)
  [Gi_1] -> combine Gi/1(Gi_1)
  cal formation tracking Gi error/1(err_Gi_form_vec) -> [err_Gi_form_vec]
  [Gi_vec] -> cal formation tracking Gi error/3(Gi_vec)
  Constant16/1 -> cal formation tracking Gi error/2(wij)
  Constant15/1 -> cal formation tracking Gi error/1(wi0)
  [dp_hat_vec] -> cal ui agent 1/6(dp_hat_vec)
  [err_Gi_form_vec] -> cal ui agent 1/3(err_Gi_form_vec)
  Constant17/1 -> cal ui agent 1/1(c_psi_p)
  [eps_p_hat_vec] -> cal ui agent 1/4(eps_p_hat_vec)
  [err_lump_vec] -> cal ui agent 1/5(err_lump_vec)
  combine ui/1(ui_vec) -> [ui]
  depart Re2/1(y) -> Display65/1
  depart Rc1/1(y) -> Display6/1
  depart Rc2/1(y) -> Display22/1
  depart Re4/1(y) -> Display67/1
  [ui] -> cal Rci from ui/2(ui)
  depart Rc5/1(y) -> Display25/1
  depart Re3/1(y) -> Display66/1
  cal Ri/1(Ri) -> [Ri]
  cal Rei/1(Rei) -> depart Re5/1(x), depart Re4/1(x), depart Re3/1(x), depart Re2/1(x), depart Re1/1(x), [Rei]
  depart Re1/1(y) -> Display64/1
  Constant51/1 -> cal Rei/1(Qei)
  [Rci] -> cal Ri/2(Rci)
  depart Re5/1(y) -> Display68/1
  [Rei] -> cal Ri/1(Rei)
  depart Rc4/1(y) -> Display24/1
  cal Rci from ui/1(Rci) -> [Rci], depart Rc5/1(x), depart Rc4/1(x), depart Rc3/1(x), depart Rc2/1(x), depart Rc1/1(x)
  depart Rc3/1(y) -> Display23/1
  Constant191/1 -> cal Rci from ui/1(mi)
  [dp_vec] -> To Workspace2/1
  [sigma_bar_v_vec] -> To Workspace12/1
  [eta_d_est_vec] -> To Workspace/1
  [eta_est_err] -> To Workspace22/1
  [sigma_v_vec] -> To Workspace19/1
  [ksi_est_err] -> To Workspace17/1
  [sigma_bar_v_tilt_vec] -> To Workspace13/1
  [dp_tilt_vec] -> To Workspace6/1
  [dp_hat_vec] -> To Workspace1/1
  [delta_ksi_vec] -> To Workspace20/1
  [ui_vec] -> To Workspace14/1
  [sigma_bar_v_hat_vec] -> To Workspace11/1
  [u0] -> To Workspace3/1
  [ksi_i_vec] -> To Workspace8/1
  [eta_i_vec] -> To Workspace7/1
  [ksi_d_est_vec] -> To Workspace18/1
  [eta0] -> To Workspace4/1
  [ksi_track_err_vec] -> To Workspace9/1
  [eta_track_err_vec] -> To Workspace10/1
  [delta_eta_vec] -> To Workspace21/1
  [ksi0] -> To Workspace5/1
  [V_init_out] -> leader eta0 Integrator/3
  Constant25/1 -> process velocity/7(R1)
  Demux1/2 -> ksi_0/2
  Demux22/2 -> eta_0/2
  Constant65/1 -> leader control input/4(R0)
  [ksi0] -> Demux1/1
  Constant24/1 -> process velocity/6(R0)
  Constant28/1 -> process velocity/9(Ry2)
  Constant68/1 -> leader control input/7(Ry2)
  Demux22/3 -> eta_0/3
  Constant70/1 -> process velocity/3(T2)
  leader eta0 Integrator/1 -> [eta0], leader ksi0 Integrator/1
  Constant29/1 -> process velocity/8(Rx2)
  Step/1 -> leader eta0 Integrator/2
  Constant73/1 -> process velocity/5(PZ1)
  Demux1/1 -> ksi_0/1
  Constant221/1 -> set desire formation configuration/7(Z1)
  Constant239/1 -> set desire formation configuration/14(T12)
  Constant30/1 -> set desire formation configuration/1(X1)
  Constant66/1 -> leader control input/5(R1)
  Constant64/1 -> leader control input/3(T2)
  Constant33/1 -> set desire formation configuration/5(Y2)
  Constant31/1 -> set desire formation configuration/2(X2)
  Constant26/1 -> process velocity/1(T0)
  Constant226/1 -> set desire formation configuration/9(Z3)
  Constant238/1 -> set desire formation configuration/13(T1)
  Constant222/1 -> set desire formation configuration/8(Z2)
  Constant69/1 -> leader control input/8(Rz2)
  Constant225/1 -> set desire formation configuration/10(theta0)
  [tsim] -> set desire formation configuration/15(t)
  Constant72/1 -> process velocity/4(PZ0)
  leader ksi0 Integrator/1 -> [ksi0]
  Constant71/1 -> process velocity/2(T1)
  Demux1/3 -> ksi_0/3
  set desire formation configuration/2(delta_eta_vec) -> [delta_eta_vec]
  Constant/1 -> leader control input/2(T1)
  [eta0] -> Demux22/1
  process velocity/1(V_init_out) -> [V_init_out]
  [u0] -> leader eta0 Integrator/1
  [delta_ksi_vec] -> desire formation position and velocity/3(delta_ksi_vec)
  desire formation position and velocity/1(pos_i_des) -> [pos_i_des]
  Constant32/1 -> set desire formation configuration/4(Y1)
  [delta_eta_vec] -> desire formation position and velocity/4(delta_eta_vec)
  Constant229/1 -> set desire formation configuration/6(Y3)
  Constant27/1 -> process velocity/10(Rz2)
  Constant67/1 -> leader control input/6(Rx2)
  [tsim] -> process velocity/11(t)
  [tsim] -> leader control input/1(t)
  set desire formation configuration/1(delta_ksi_vec) -> [delta_ksi_vec]
  Constant235/1 -> set desire formation configuration/12(kai_3_t)
  Clock/1 -> [tsim]
  desire formation position and velocity/2(vel_i_des) -> [vel_i_des]
  [eta0] -> desire formation position and velocity/2(eta0)
  [ksi0] -> desire formation position and velocity/1(ksi0)
  Demux22/1 -> eta_0/1
  Constant234/1 -> set desire formation configuration/3(X3)
  Constant231/1 -> set desire formation configuration/11(kai_1_t)
  leader control input/1(u0) -> [u0]
  trans to column57/1(y) -> [eta_est_err_squ_2_node_4], Display91/1
  Demux73/1 -> Mux99/1
  trans to column44/1(y) -> [ksi_est_err_squ_1_node_2], Display79/1
  Demux78/1 -> Mux86/1
  Mux94/1 -> eta_d_est_1/3
  cal theta_eta_est_err_tilt agent 5/1(theta_eta_est_err_tilt_1_5) -> [theta_eta_est_err_tilt_1_5]
  choose eta_est_err_tilt 1/1(y) -> cal abs 41/1(x)
  Demux76/1 -> Mux102/2
  Constant265/1 -> Mux117/2
  Constant266/1 -> Mux117/3
  cal theta_eta_est_err_tilt agent 3/2(theta_eta_est_err_tilt_2_3) -> [theta_eta_est_err_tilt_2_3]
  Demux72/2 -> Mux96/2
  [theta_ksi_est_err_tilt_2_5] -> combine lumped follower position observation error/10(theta_ksi_est_err_tilt_2_5)
  Constant259/1 -> Mux116/3
  [theta_eta_est_err_tilt_2_vec] -> fixed-time distributed follower desire velocity observer agent 2/4(theta_eta_est_err_tilt_2_vec)
  cal abs 45/1(y) -> Mux120/1
  fixed-time distributed follower desire velocity observer agent 2/1(d_eta_d_est_2) -> velocity observe Integrator 2/1
  Add/1 -> Demux70/1
  Demux72/1 -> Mux95/2
  Mux95/1 -> eta_d_est_2/1
  velocity observe Integrator 2/1 -> [eta_d_est_2], Demux71/1
  Demux76/3 -> Mux104/2
  Constant281/1 -> Mux128/2
  Demux77/1 -> Mux105/1
  Mux103/1 -> eta_d_est_4/2
  [eta_d_est_4] -> combine follower desire velocity estimaters/4(eta_d_est_4)
  [theta_eta_est_err_tilt_2_5] -> combine lumped follower velocity observation error/10(theta_eta_est_err_tilt_2_5)
  trans to column51/1(y) -> [ksi_est_err_squ_1_node_5], Display86/1
  [eta_est_err_tilt_vec] -> cal theta_eta_est_err_tilt agent 4/4(eta_est_err_tilt_vec)
  [theta_ksi_est_err_tilt_2_4] -> combine lumped follower position observation error/9(theta_ksi_est_err_tilt_2_4)
  [eta_est_err_tilt_vec] -> cal theta_eta_est_err_tilt agent 2/4(eta_est_err_tilt_vec)
  [ksi_est_err_tilt_vec] -> choose eta_est_err_tilt 18/1(x)
  Mux113/1 -> Interpreted MATLAB Function56/1
  Add6/1 -> Demux93/1
  Demux93/1 -> Mux119/2
  choose eta_est_err_tilt 18/1(y) -> cal abs 50/1(x)
  [ksi_est_err_squ_1_node_3] -> cal theta_ksi_est_err_tilt agent 3/2(ksi_est_err_squ_1_node_3)
  Constant252/1 -> fixed-time distributed follower desire position observer agent 3/2(l2p)
  Constant203/1 -> fixed-time distributed follower desire velocity observer agent 2/1(l1v)
  Add8/1 -> Demux97/1
  [eta_est_err_squ_1_node_2] -> cal theta_eta_est_err_tilt agent 2/2(eta_est_err_squ_1_node_2)
  Add3/1 -> Demux76/1
  [eta_est_err_squ_1_node_3] -> cal theta_eta_est_err_tilt agent 3/2(eta_est_err_squ_1_node_3)
  Constant200/1 -> fixed-time distributed follower desire velocity observer agent 1/1(l1v)
  cal abs 43/1(y) -> Mux126/1
  choose eta_est_err_tilt 16/1(y) -> cal abs 48/1(x)
  Interpreted MATLAB Function47/1 -> trans to column47/1(x)
  Constant261/1 -> Mux114/3
  choose eta_est_err_tilt 14/1(y) -> cal abs 46/1(x)
  [ksi_est_err_tilt_vec] -> choose eta_est_err_tilt 19/1(x)
  position observe Integrator 4/1 -> [ksi_d_est_4], Demux96/1
  [theta_eta_est_err_tilt_1_1] -> combine lumped follower velocity observation error/1(theta_eta_est_err_tilt_1_1)
  Constant280/1 -> Mux129/3
  Mux108/1 -> ksi_d_est_1/3
  [eta_est_err_squ_2_node_5] -> cal theta_eta_est_err_tilt agent 5/3(eta_est_err_squ_2_node_5)
  Mux90/1 -> ksi_d_est_5/1
  cal theta_ksi_est_err_tilt agent 4/2(theta_ksi_est_err_tilt_2_4) -> [theta_ksi_est_err_tilt_2_4]
  [eta_d_est_2] -> combine follower desire velocity estimaters/2(eta_d_est_2)
  Constant187/1 -> fixed-time distributed follower desire position observer agent 4/1(l1p)
  Demux69/3 -> Mux94/1
  [ksi0] -> Add9/1
  [ksi0] -> Add7/1
  [theta_eta_est_err_tilt_2_vec] -> fixed-time distributed follower desire velocity observer agent 5/4(theta_eta_est_err_tilt_2_vec)
  Constant189/1 -> fixed-time distributed follower desire position observer agent 5/2(l2p)
  Interpreted MATLAB Function45/1 -> trans to column45/1(x)
  [theta_ksi_est_err_tilt_1_vec] -> fixed-time distributed follower desire position observer agent 2/4(theta_ksi_est_err_tilt_1_vec)
  Demux71/2 -> Mux96/1
  [theta_ksi_est_err_tilt_2_vec] -> fixed-time distributed follower desire position observer agent 2/5(theta_ksi_est_err_tilt_2_vec)
  fixed-time distributed follower desire position observer agent 5/1(d_ksi_d_est_5) -> position observe Integrator 5/1
  [theta_ksi_est_err_tilt_2_vec] -> fixed-time distributed follower desire position observer agent 1/5(theta_ksi_est_err_tilt_2_vec)
  cal theta_ksi_est_err_tilt agent 5/1(theta_ksi_est_err_tilt_1_5) -> [theta_ksi_est_err_tilt_1_5]
  Mux135/1 -> ksi_d_est_3/3
  position observe Integrator 3/1 -> [ksi_d_est_3], Demux94/1
  [theta_ksi_est_err_tilt_1_4] -> combine lumped follower position observation error/4(theta_ksi_est_err_tilt_1_4)
  [ksi_d_est_5] -> combine leader position estimaters/5(ksi_d_est_5)
  [theta_ksi_est_err_tilt_1_3] -> combine lumped follower position observation error/3(theta_ksi_est_err_tilt_1_3)
  Mux118/1 -> Interpreted MATLAB Function60/1
  Constant197/1 -> fixed-time distributed follower desire position observer agent 1/1(l1p)
  [eta_est_err_tilt_vec] -> choose eta_est_err_tilt 10/1(x)
  Mux120/1 -> Interpreted MATLAB Function42/1
  [theta_eta_est_err_tilt_1_3] -> combine lumped follower velocity observation error/3(theta_eta_est_err_tilt_1_3)
  cal abs 50/1(y) -> Mux127/1
  Mux109/1 -> Interpreted MATLAB Function41/1
  fixed-time distributed follower desire velocity observer agent 5/1(d_eta_d_est_5) -> velocity observe Integrator 5/1
  cal abs 58/1(y) -> Mux116/1
  Interpreted MATLAB Function60/1 -> trans to column60/1(x)
  Constant262/1 -> Mux118/2
  choose eta_est_err_tilt 7/1(y) -> cal abs 58/1(x)
  Constant282/1 -> Mux128/3
  cal theta_ksi_est_err_tilt agent 1/1(theta_ksi_est_err_tilt_1_1) -> [theta_ksi_est_err_tilt_1_1]
  Constant208/1 -> Add5/2
  Interpreted MATLAB Function58/1 -> trans to column58/1(x)
  Mux107/1 -> eta_d_est_5/3
  Mux130/1 -> ksi_d_est_2/2
  position observe Integrator 1/1 -> [ksi_d_est_1], Demux78/1
  [ksi_est_err_squ_2_node_5] -> cal theta_ksi_est_err_tilt agent 5/3(ksi_est_err_squ_2_node_5)
  [ksi_est_err_tilt_vec] -> choose eta_est_err_tilt 13/1(x)
  Constant254/1 -> Mux113/2
  Demux88/2 -> Mux97/2
  Constant278/1 -> Mux125/3
  [theta_ksi_est_err_tilt_1_5] -> combine lumped follower position observation error/5(theta_ksi_est_err_tilt_1_5)
  Constant185/1 -> cal theta_ksi_est_err_tilt agent 4/1(alfa_theta)
  Constant247/1 -> Mux109/2
  Constant207/1 -> Add2/2
  [eta_est_err_squ_2_node_2] -> cal theta_eta_est_err_tilt agent 2/3(eta_est_err_squ_2_node_2)
  choose eta_est_err_tilt 8/1(y) -> cal abs 59/1(x)
  Constant182/1 -> fixed-time distributed follower desire position observer agent 1/2(l2p)
  Mux98/1 -> eta_d_est_2/3
  [ksi_est_err_tilt_vec] -> choose eta_est_err_tilt 16/1(x)
  [eta_est_err_tilt_vec] -> choose eta_est_err_tilt 6/1(x)
  combine lumped follower position observation error/2(theta_ksi_est_err_tilt_2_vec) -> [theta_ksi_est_err_tilt_2_vec]
  Mux111/1 -> Interpreted MATLAB Function53/1
  choose eta_est_err_tilt 4/1(y) -> cal abs 55/1(x)
  Demux92/3 -> Mux132/1
  Constant253/1 -> Mux110/3
  Mux86/1 -> ksi_d_est_1/1
  [eta_d_est_vec] -> fixed-time distributed follower desire position observer agent 1/3(eta_d_est_vec)
  Mux92/1 -> eta_d_est_1/1
  choose eta_est_err_tilt 15/1(y) -> cal abs 47/1(x)
  [eta_est_err_tilt_vec] -> choose eta_est_err_tilt 4/1(x)
  [ksi_est_err_tilt_vec] -> choose eta_est_err_tilt 17/1(x)
  Mux125/1 -> Interpreted MATLAB Function48/1
  [theta_eta_est_err_tilt_2_2] -> combine lumped follower velocity observation error/7(theta_eta_est_err_tilt_2_2)
  choose eta_est_err_tilt 2/1(y) -> cal abs 52/1(x)
  Constant184/1 -> cal theta_ksi_est_err_tilt agent 3/1(alfa_theta)
  [theta_ksi_est_err_tilt_1_vec] -> fixed-time distributed follower desire position observer agent 1/4(theta_ksi_est_err_tilt_1_vec)
  Constant193/1 -> cal theta_eta_est_err_tilt agent 1/1(alfa_theta)
  Interpreted MATLAB Function54/1 -> trans to column54/1(x)
  Constant188/1 -> Add8/2
  Constant277/1 -> Mux125/2
  [eta_est_err_squ_2_node_1] -> cal theta_eta_est_err_tilt agent 1/3(eta_est_err_squ_2_node_1)
  Constant199/1 -> fixed-time distributed follower desire velocity observer agent 1/2(l2v)
  [theta_eta_est_err_tilt_1_vec] -> fixed-time distributed follower desire velocity observer agent 3/3(theta_eta_est_err_tilt_1_vec)
  [ksi_est_err_tilt_vec] -> choose eta_est_err_tilt 12/1(x)
  Mux105/1 -> eta_d_est_5/1
  Mux128/1 -> Interpreted MATLAB Function50/1
  [ksi_est_err_squ_2_node_2] -> cal theta_ksi_est_err_tilt agent 2/3(ksi_est_err_squ_2_node_2)
  cal abs 47/1(y) -> Mux121/1
  Demux70/1 -> Mux92/2
  Constant276/1 -> Mux127/3
  Constant218/1 -> Mux120/3
  [ksi_d_est_1] -> combine leader position estimaters/1(ksi_d_est_1)
  Constant263/1 -> fixed-time distributed follower desire position observer agent 3/1(l1p)
  Constant270/1 -> Mux124/2
  trans to column42/1(y) -> [ksi_est_err_squ_2_node_1], Display77/1
  Interpreted MATLAB Function44/1 -> trans to column44/1(x)
  Constant245/1 -> Mux115/2
  Constant249/1 -> Mux111/2
  Add1/1 -> Demux72/1
  Demux95/1 -> Mux133/2
  cal abs 49/1(y) -> Mux123/1
  [theta_eta_est_err_tilt_1_vec] -> fixed-time distributed follower desire velocity observer agent 2/3(theta_eta_est_err_tilt_1_vec)
  choose eta_est_err_tilt 17/1(y) -> cal abs 49/1(x)
  choose eta_est_err_tilt 20/1(y) -> cal abs 53/1(x)
  Demux78/3 -> Mux108/1
  Constant201/1 -> Add/2
  Demux78/2 -> Mux97/1
  Constant205/1 -> fixed-time distributed follower desire velocity observer agent 3/2(l2v)
  [ksi0] -> Add6/1
  Demux72/3 -> Mux98/2
  Mux97/1 -> ksi_d_est_1/2
  Constant194/1 -> cal theta_eta_est_err_tilt agent 2/1(alfa_theta)
  trans to column52/1(y) -> [eta_est_err_squ_2_node_2], Display87/1
  [theta_eta_est_err_tilt_1_vec] -> fixed-time distributed follower desire velocity observer agent 5/3(theta_eta_est_err_tilt_1_vec)
  cal theta_eta_est_err_tilt agent 1/1(theta_eta_est_err_tilt_1_1) -> [theta_eta_est_err_tilt_1_1]
  fixed-time distributed follower desire position observer agent 2/1(d_ksi_d_est_2) -> position observe Integrator 2/1
  Mux116/1 -> Interpreted MATLAB Function58/1
  Mux131/1 -> ksi_d_est_5/3
  Add7/1 -> Demux95/1
  [ksi_est_err_squ_1_node_5] -> cal theta_ksi_est_err_tilt agent 5/2(ksi_est_err_squ_1_node_5)
  Demux69/1 -> Mux92/1
  Demux95/2 -> Mux134/2
  Constant258/1 -> Mux116/2
  [eta_est_err_tilt_vec] -> choose eta_est_err_tilt 9/1(x)
  fixed-time distributed follower desire position observer agent 1/1(d_ksi_d_est_1) -> position observe Integrator 1/1
  cal theta_ksi_est_err_tilt agent 5/2(theta_ksi_est_err_tilt_2_5) -> [theta_ksi_est_err_tilt_2_5]
  Demux69/2 -> Mux93/1
  Constant275/1 -> Mux127/2
  cal abs 59/1(y) -> Mux114/1
  [ksi_est_err_tilt_vec] -> choose eta_est_err_tilt 20/1(x)
  choose eta_est_err_tilt 13/1(y) -> cal abs 45/1(x)
  choose eta_est_err_tilt 9/1(y) -> cal abs 60/1(x)
  Mux100/1 -> eta_d_est_3/2
  Constant274/1 -> Add7/2
  [ksi_est_err_squ_2_node_3] -> cal theta_ksi_est_err_tilt agent 3/3(ksi_est_err_squ_2_node_3)
  [eta_d_est_vec] -> fixed-time distributed follower desire position observer agent 3/3(eta_d_est_vec)
  Constant257/1 -> Mux112/3
  cal theta_eta_est_err_tilt agent 4/1(theta_eta_est_err_tilt_1_4) -> [theta_eta_est_err_tilt_1_4]
  Demux77/3 -> Mux107/1
  [eta_est_err_tilt_vec] -> choose eta_est_err_tilt 7/1(x)
  [ksi_est_err_squ_2_node_4] -> cal theta_ksi_est_err_tilt agent 4/3(ksi_est_err_squ_2_node_4)
  Demux74/3 -> Mux101/2
  [theta_ksi_est_err_tilt_2_vec] -> fixed-time distributed follower desire position observer agent 5/5(theta_ksi_est_err_tilt_2_vec)
  Demux68/2 -> Mux91/1
  [eta0] -> Add/1
  [ksi_est_err_tilt_vec] -> cal theta_ksi_est_err_tilt agent 5/4(ksi_est_err_tilt_vec)
  cal theta_eta_est_err_tilt agent 5/2(theta_eta_est_err_tilt_2_5) -> [theta_eta_est_err_tilt_2_5]
  Demux77/2 -> Mux106/1
  Constant219/1 -> fixed-time distributed follower desire position observer agent 2/2(l2p)
  [eta_est_err_tilt_vec] -> choose eta_est_err_tilt 8/1(x)
  velocity observe Integrator 3/1 -> [eta_d_est_3], Demux73/1
  Interpreted MATLAB Function57/1 -> trans to column57/1(x)
  cal abs 53/1(y) -> Mux129/1
  Mux87/1 -> ksi_d_est_4/1
  cal abs 44/1(y) -> Mux128/1
  [theta_ksi_est_err_tilt_2_3] -> combine lumped follower position observation error/8(theta_ksi_est_err_tilt_2_3)
  Demux80/3 -> Mux131/2
  Demux75/1 -> Mux102/1
  Constant248/1 -> Mux109/3
  Constant215/1 -> Mux126/2
  Mux121/1 -> Interpreted MATLAB Function43/1
  fixed-time distributed follower desire velocity observer agent 4/1(d_eta_d_est_4) -> velocity observe Integrator 4/1
  Demux94/3 -> Mux135/1
  cal abs 42/1(y) -> Mux117/1
  [theta_ksi_est_err_tilt_2_2] -> combine lumped follower position observation error/7(theta_ksi_est_err_tilt_2_2)
  Mux93/1 -> eta_d_est_1/2
  [ksi_est_err_squ_1_node_2] -> cal theta_ksi_est_err_tilt agent 2/2(ksi_est_err_squ_1_node_2)
  [ksi0] -> Add8/1
  velocity observe Integrator 5/1 -> [eta_d_est_5], Demux77/1
  combine lumped follower velocity observation error/2(theta_eta_est_err_tilt_2_vec) -> [theta_eta_est_err_tilt_2_vec]
  [ksi_est_err_squ_1_node_4] -> cal theta_ksi_est_err_tilt agent 4/2(ksi_est_err_squ_1_node_4)
  [eta_est_err_tilt_vec] -> cal theta_eta_est_err_tilt agent 3/4(eta_est_err_tilt_vec)
  Demux95/3 -> Mux135/2
  choose eta_est_err_tilt 12/1(y) -> cal abs 44/1(x)
  combine follower desire velocity estimaters/1(eta_d_est_vec) -> [eta_d_est_vec]
  Constant272/1 -> Mux123/2
  [eta_d_est_vec] -> fixed-time distributed follower desire position observer agent 5/3(eta_d_est_vec)
  Mux106/1 -> eta_d_est_5/2
  [theta_eta_est_err_tilt_1_4] -> combine lumped follower velocity observation error/4(theta_eta_est_err_tilt_1_4)
  cal abs 41/1(y) -> Mux115/1
  [eta_d_est_1] -> combine follower desire velocity estimaters/1(eta_d_est_1)
  Constant264/1 -> Mux118/3
  choose eta_est_err_tilt 6/1(y) -> cal abs 57/1(x)
  Demux70/2 -> Mux93/2
  [ksi_est_err_tilt_vec] -> cal theta_ksi_est_err_tilt agent 1/4(ksi_est_err_tilt_vec)
  Constant214/1 -> Add4/2
  Mux126/1 -> Interpreted MATLAB Function45/1
  [ksi0] -> Add5/1
  Interpreted MATLAB Function42/1 -> trans to column42/1(x)
  Interpreted MATLAB Function49/1 -> trans to column49/1(x)
  Interpreted MATLAB Function43/1 -> trans to column43/1(x)
  Constant256/1 -> Mux112/2
  trans to column53/1(y) -> [eta_est_err_squ_1_node_2], Display88/1
  Mux114/1 -> Interpreted MATLAB Function57/1
  [eta_est_err_tilt_vec] -> choose eta_est_err_tilt 3/1(x)
  Interpreted MATLAB Function51/1 -> trans to column51/1(x)
  Constant202/1 -> fixed-time distributed follower desire velocity observer agent 2/2(l2v)
  cal abs 48/1(y) -> Mux124/1
  [theta_eta_est_err_tilt_2_1] -> combine lumped follower velocity observation error/6(theta_eta_est_err_tilt_2_1)
  Mux124/1 -> Interpreted MATLAB Function47/1
  Constant283/1 -> cal theta_ksi_est_err_tilt agent 1/1(alfa_theta)
  cal abs 57/1(y) -> Mux112/1
  cal theta_eta_est_err_tilt agent 1/2(theta_eta_est_err_tilt_2_1) -> [theta_eta_est_err_tilt_2_1]
  [eta_est_err_tilt_vec] -> cal theta_eta_est_err_tilt agent 5/4(eta_est_err_tilt_vec)
  Constant195/1 -> cal theta_eta_est_err_tilt agent 3/1(alfa_theta)
  Mux89/1 -> ksi_d_est_4/3
  trans to column45/1(y) -> [ksi_est_err_squ_1_node_1], Display84/1
  Mux132/1 -> ksi_d_est_2/3
  Add9/1 -> Demux80/1
  Constant260/1 -> Mux114/2
  Demux68/1 -> Mux90/1
  [ksi_est_err_tilt_vec] -> cal theta_ksi_est_err_tilt agent 4/4(ksi_est_err_tilt_vec)
  Mux102/1 -> eta_d_est_4/1
  [theta_eta_est_err_tilt_1_vec] -> fixed-time distributed follower desire velocity observer agent 1/3(theta_eta_est_err_tilt_1_vec)
  Interpreted MATLAB Function50/1 -> trans to column50/1(x)
  Add4/1 -> Demux79/1
  Interpreted MATLAB Function48/1 -> trans to column48/1(x)
  Interpreted MATLAB Function53/1 -> trans to column53/1(x)
  Constant284/1 -> cal theta_ksi_est_err_tilt agent 2/1(alfa_theta)
  fixed-time distributed follower desire velocity observer agent 1/1(d_eta_d_est_1) -> velocity observe Integrator 1/1
  Interpreted MATLAB Function56/1 -> trans to column56/1(x)
  [theta_eta_est_err_tilt_2_vec] -> fixed-time distributed follower desire velocity observer agent 1/4(theta_eta_est_err_tilt_2_vec)
  Demux68/3 -> Mux131/1
  trans to column50/1(y) -> [ksi_est_err_squ_2_node_5], Display85/1
  cal theta_ksi_est_err_tilt agent 3/2(theta_ksi_est_err_tilt_2_3) -> [theta_ksi_est_err_tilt_2_3]
  [eta_est_err_squ_1_node_1] -> cal theta_eta_est_err_tilt agent 1/2(eta_est_err_squ_1_node_1)
  trans to column48/1(y) -> [ksi_est_err_squ_2_node_4], Display82/1
  trans to column43/1(y) -> [ksi_est_err_squ_2_node_2], Display78/1
  [ksi_d_est_3] -> combine leader position estimaters/3(ksi_d_est_3)
  Demux92/1 -> Mux119/1
  Constant192/1 -> Add9/2
  [eta0] -> Add3/1
  Mux101/1 -> eta_d_est_3/3
  combine lumped follower velocity observation error/1(theta_eta_est_err_tilt_1_vec) -> [theta_eta_est_err_tilt_1_vec]
  Mux119/1 -> ksi_d_est_2/1
  Mux127/1 -> Interpreted MATLAB Function49/1
  [theta_ksi_est_err_tilt_1_vec] -> fixed-time distributed follower desire position observer agent 4/4(theta_ksi_est_err_tilt_1_vec)
  [eta_d_est_3] -> combine follower desire velocity estimaters/3(eta_d_est_3)
  Demux79/2 -> Mux106/2
  cal theta_ksi_est_err_tilt agent 2/1(theta_ksi_est_err_tilt_1_2) -> [theta_ksi_est_err_tilt_1_2]
  [ksi_d_est_4] -> combine leader position estimaters/4(ksi_d_est_4)
  Demux76/2 -> Mux103/2
  [theta_eta_est_err_tilt_1_5] -> combine lumped follower velocity observation error/5(theta_eta_est_err_tilt_1_5)
  Mux91/1 -> ksi_d_est_5/2
  cal abs 54/1(y) -> Mux111/1
  cal abs 52/1(y) -> Mux109/1
  Demux79/3 -> Mux107/2
  velocity observe Integrator 1/1 -> [eta_d_est_1], Demux69/1
  cal theta_eta_est_err_tilt agent 2/1(theta_eta_est_err_tilt_1_2) -> [theta_eta_est_err_tilt_1_2]
  position observe Integrator 2/1 -> [ksi_d_est_2], Demux92/1
  Mux117/1 -> Interpreted MATLAB Function59/1
  Demux80/1 -> Mux90/2
  Mux96/1 -> eta_d_est_2/2
  Demux97/3 -> Mux89/2
  position observe Integrator 5/1 -> [ksi_d_est_5], Demux68/1
  Interpreted MATLAB Function52/1 -> trans to column52/1(x)
  [theta_eta_est_err_tilt_2_vec] -> fixed-time distributed follower desire velocity observer agent 3/4(theta_eta_est_err_tilt_2_vec)
  Constant211/1 -> Add3/2
  Demux71/3 -> Mux98/1
  cal abs 56/1(y) -> Mux113/1
  Constant255/1 -> Mux113/3
  [eta_est_err_squ_1_node_5] -> cal theta_eta_est_err_tilt agent 5/2(eta_est_err_squ_1_node_5)
  [theta_eta_est_err_tilt_2_4] -> combine lumped follower velocity observation error/9(theta_eta_est_err_tilt_2_4)
  [eta0] -> Add2/1
  Demux80/2 -> Mux91/2
  choose eta_est_err_tilt 5/1(y) -> cal abs 56/1(x)
  Demux96/1 -> Mux87/1
  Mux104/1 -> eta_d_est_4/3
  [theta_ksi_est_err_tilt_2_vec] -> fixed-time distributed follower desire position observer agent 3/5(theta_ksi_est_err_tilt_2_vec)
  Demux96/2 -> Mux88/1
  Constant213/1 -> fixed-time distributed follower desire velocity observer agent 5/1(l1v)
  Mux88/1 -> ksi_d_est_4/2
  Add5/1 -> Demux88/1
  [eta_d_est_vec] -> fixed-time distributed follower desire position observer agent 2/3(eta_d_est_vec)
  Constant206/1 -> fixed-time distributed follower desire velocity observer agent 3/1(l1v)
  Constant183/1 -> fixed-time distributed follower desire position observer agent 4/2(l2p)
  trans to column41/1(y) -> [eta_est_err_squ_2_node_1], Display76/1
  Demux94/2 -> Mux134/1
  choose eta_est_err_tilt 10/1(y) -> cal abs 42/1(x)
  Constant196/1 -> cal theta_eta_est_err_tilt agent 4/1(alfa_theta)
  [theta_ksi_est_err_tilt_1_2] -> combine lumped follower position observation error/2(theta_ksi_est_err_tilt_1_2)
  [eta_est_err_squ_2_node_4] -> cal theta_eta_est_err_tilt agent 4/3(eta_est_err_squ_2_node_4)
  combine lumped follower position observation error/1(theta_ksi_est_err_tilt_1_vec) -> [theta_ksi_est_err_tilt_1_vec]
  Demux75/3 -> Mux104/1
  Constant230/1 -> fixed-time distributed follower desire position observer agent 2/1(l1p)
  [eta_est_err_tilt_vec] -> cal theta_eta_est_err_tilt agent 1/4(eta_est_err_tilt_vec)
  cal abs 51/1(y) -> Mux125/1
  [theta_eta_est_err_tilt_2_vec] -> fixed-time distributed follower desire velocity observer agent 4/4(theta_eta_est_err_tilt_2_vec)
  fixed-time distributed follower desire velocity observer agent 3/1(d_eta_d_est_3) -> velocity observe Integrator 3/1
  Demux97/1 -> Mux87/2
  Mux134/1 -> ksi_d_est_3/2
  Add2/1 -> Demux74/1
  cal theta_ksi_est_err_tilt agent 2/2(theta_ksi_est_err_tilt_2_2) -> [theta_ksi_est_err_tilt_2_2]
  [ksi_est_err_squ_2_node_1] -> cal theta_ksi_est_err_tilt agent 1/3(ksi_est_err_squ_2_node_1)
  Constant241/1 -> Add6/2
  [eta0] -> Add4/1
  Constant204/1 -> Add1/2
  Constant269/1 -> Mux121/3
  [theta_ksi_est_err_tilt_1_vec] -> fixed-time distributed follower desire position observer agent 5/4(theta_ksi_est_err_tilt_1_vec)
  Constant251/1 -> Mux110/2
  Constant273/1 -> Mux123/3
  Mux115/1 -> Interpreted MATLAB Function54/1
  Interpreted MATLAB Function41/1 -> trans to column41/1(x)
  Constant217/1 -> Mux120/2
  Constant271/1 -> Mux124/3
  [eta_d_est_5] -> combine follower desire velocity estimaters/5(eta_d_est_5)
  [ksi_est_err_tilt_vec] -> choose eta_est_err_tilt 15/1(x)
  cal theta_ksi_est_err_tilt agent 3/1(theta_ksi_est_err_tilt_1_3) -> [theta_ksi_est_err_tilt_1_3]
  [ksi_est_err_tilt_vec] -> choose eta_est_err_tilt 11/1(x)
  [eta0] -> Add1/1
  fixed-time distributed follower desire position observer agent 4/1(d_ksi_d_est_4) -> position observe Integrator 4/1
  choose eta_est_err_tilt 3/1(y) -> cal abs 54/1(x)
  [theta_eta_est_err_tilt_2_3] -> combine lumped follower velocity observation error/8(theta_eta_est_err_tilt_2_3)
  [theta_ksi_est_err_tilt_1_1] -> combine lumped follower position observation error/1(theta_ksi_est_err_tilt_1_1)
  Demux92/2 -> Mux130/1
  [eta_est_err_squ_2_node_3] -> cal theta_eta_est_err_tilt agent 3/3(eta_est_err_squ_2_node_3)
  Mux133/1 -> ksi_d_est_3/1
  [ksi_est_err_squ_1_node_1] -> cal theta_ksi_est_err_tilt agent 1/2(ksi_est_err_squ_1_node_1)
  cal theta_ksi_est_err_tilt agent 1/2(theta_ksi_est_err_tilt_2_1) -> [theta_ksi_est_err_tilt_2_1]
  [eta_est_err_tilt_vec] -> choose eta_est_err_tilt 5/1(x)
  [ksi_est_err_tilt_vec] -> cal theta_ksi_est_err_tilt agent 2/4(ksi_est_err_tilt_vec)
  Demux70/3 -> Mux94/2
  Constant212/1 -> fixed-time distributed follower desire velocity observer agent 5/2(l2v)
  Mux123/1 -> Interpreted MATLAB Function46/1
  Demux74/1 -> Mux99/2
  trans to column56/1(y) -> [eta_est_err_squ_1_node_3], Display90/1
  Constant209/1 -> fixed-time distributed follower desire velocity observer agent 4/2(l2v)
  Demux93/3 -> Mux132/2
  Constant190/1 -> fixed-time distributed follower desire position observer agent 5/1(l1p)
  cal theta_eta_est_err_tilt agent 4/2(theta_eta_est_err_tilt_2_4) -> [theta_eta_est_err_tilt_2_4]
  Mux99/1 -> eta_d_est_3/1
  Constant216/1 -> Mux126/3
  Mux122/1 -> Interpreted MATLAB Function44/1
  choose eta_est_err_tilt 19/1(y) -> cal abs 51/1(x)
  Interpreted MATLAB Function59/1 -> trans to column59/1(x)
  [eta_est_err_squ_1_node_4] -> cal theta_eta_est_err_tilt agent 4/2(eta_est_err_squ_1_node_4)
  [theta_ksi_est_err_tilt_2_1] -> combine lumped follower position observation error/6(theta_ksi_est_err_tilt_2_1)
  fixed-time distributed follower desire position observer agent 3/1(d_ksi_d_est_3) -> position observe Integrator 3/1
  Demux88/3 -> Mux108/2
  choose eta_est_err_tilt 11/1(y) -> cal abs 43/1(x)
  Demux93/2 -> Mux130/2
  Demux75/2 -> Mux103/1
  trans to column49/1(y) -> [ksi_est_err_squ_1_node_4], Display83/1
  Demux79/1 -> Mux105/2
  [ksi_d_est_2] -> combine leader position estimaters/2(ksi_d_est_2)
  trans to column58/1(y) -> [eta_est_err_squ_1_node_4], Display92/1
  [eta_est_err_tilt_vec] -> choose eta_est_err_tilt 1/1(x)
  Demux74/2 -> Mux100/2
  trans to column46/1(y) -> [ksi_est_err_squ_2_node_3], Display80/1
  cal theta_ksi_est_err_tilt agent 4/1(theta_ksi_est_err_tilt_1_4) -> [theta_ksi_est_err_tilt_1_4]
  [ksi_est_err_tilt_vec] -> cal theta_ksi_est_err_tilt agent 3/4(ksi_est_err_tilt_vec)
  Demux73/2 -> Mux100/1
  combine leader position estimaters/1(ksi_d_est_vec) -> [ksi_d_est_vec]
  [ksi_est_err_tilt_vec] -> choose eta_est_err_tilt 14/1(x)
  trans to column59/1(y) -> [eta_est_err_squ_2_node_5], Display94/1
  [eta_d_est_vec] -> fixed-time distributed follower desire position observer agent 4/3(eta_d_est_vec)
  cal theta_eta_est_err_tilt agent 3/1(theta_eta_est_err_tilt_1_3) -> [theta_eta_est_err_tilt_1_3]
  Constant268/1 -> Mux121/2
  [eta_est_err_tilt_vec] -> choose eta_est_err_tilt 2/1(x)
  Constant250/1 -> Mux111/3
  Constant198/1 -> cal theta_eta_est_err_tilt agent 5/1(alfa_theta)
  Interpreted MATLAB Function46/1 -> trans to column46/1(x)
  Demux96/3 -> Mux89/1
  Constant246/1 -> Mux115/3
  trans to column60/1(y) -> [eta_est_err_squ_1_node_5], Display95/1
  Constant186/1 -> cal theta_ksi_est_err_tilt agent 5/1(alfa_theta)
  [theta_eta_est_err_tilt_1_vec] -> fixed-time distributed follower desire velocity observer agent 4/3(theta_eta_est_err_tilt_1_vec)
  Mux129/1 -> Interpreted MATLAB Function51/1
  trans to column47/1(y) -> [ksi_est_err_squ_1_node_3], Display81/1
  [theta_ksi_est_err_tilt_1_vec] -> fixed-time distributed follower desire position observer agent 3/4(theta_ksi_est_err_tilt_1_vec)
  Demux94/1 -> Mux133/1
  trans to column55/1(y) -> [eta_est_err_squ_2_node_3], Display89/1
  Mux112/1 -> Interpreted MATLAB Function55/1
  Constant279/1 -> Mux129/2
  [theta_eta_est_err_tilt_1_2] -> combine lumped follower velocity observation error/2(theta_eta_est_err_tilt_1_2)
  Demux71/1 -> Mux95/1
  Mux110/1 -> Interpreted MATLAB Function52/1
  cal abs 55/1(y) -> Mux110/1
  Interpreted MATLAB Function55/1 -> trans to column55/1(x)
  velocity observe Integrator 4/1 -> [eta_d_est_4], Demux75/1
  Demux73/3 -> Mux101/1
  [theta_ksi_est_err_tilt_2_vec] -> fixed-time distributed follower desire position observer agent 4/5(theta_ksi_est_err_tilt_2_vec)
  cal abs 46/1(y) -> Mux122/1
  Demux97/2 -> Mux88/2
  cal abs 60/1(y) -> Mux118/1
  Constant220/1 -> Mux122/2
  trans to column54/1(y) -> [eta_est_err_squ_1_node_1], Display93/1
  cal theta_eta_est_err_tilt agent 2/2(theta_eta_est_err_tilt_2_2) -> [theta_eta_est_err_tilt_2_2]
  Constant210/1 -> fixed-time distributed follower desire velocity observer agent 4/1(l1v)
  Demux88/1 -> Mux86/2
  Constant267/1 -> Mux122/3
  cal lumped observation error agent 3/1(ksi_est_err_tilt_3) -> [ksi_est_err_tilt_3]
  [ksi_d_est_vec] -> cal lumped observation error agent 5/3(ksi_d_est_vec)
  cal lumped observation error agent 5/1(ksi_est_err_tilt_5) -> [ksi_est_err_tilt_5]
  Constant227/1 -> cal lumped observation error agent 2/1(wij)
  Constant232/1 -> cal lumped observation error agent 3/1(wij)
  [ksi_est_err_tilt_5] -> "combine lumped follower observation error "/5(ksi_est_err_tilt_5)
  [ksi0] -> cal lumped observation error agent 3/4(ksi0)
  [ksi0] -> cal lumped observation error agent 1/4(ksi0)
  Constant236/1 -> cal lumped observation error agent 4/1(wij)
  "combine lumped follower observation error "/2(eta_est_err_tilt_vec) -> [eta_est_err_tilt_vec]
  cal lumped observation error agent 5/2(eta_est_err_tilt_5) -> [eta_est_err_tilt_5]
  [eta_d_est_vec] -> cal lumped observation error agent 4/6(eta_d_est_vec)
  [ksi0] -> cal lumped observation error agent 4/4(ksi0)
  Constant224/1 -> cal lumped observation error agent 1/2(w0)
  [delta_eta_vec] -> cal lumped observation error agent 4/8(delta_eta_vec)
  [delta_ksi_vec] -> cal lumped observation error agent 4/5(delta_ksi_vec)
  [eta_est_err_tilt_3] -> "combine lumped follower observation error "/8(eta_est_err_tilt_3)
  [eta_d_est_vec] -> cal lumped observation error agent 2/6(eta_d_est_vec)
  [delta_ksi_vec] -> cal lumped observation error agent 2/5(delta_ksi_vec)
  [ksi_est_err_tilt_4] -> "combine lumped follower observation error "/4(ksi_est_err_tilt_4)
  [delta_ksi_vec] -> cal lumped observation error agent 1/5(delta_ksi_vec)
  [eta0] -> cal lumped observation error agent 5/7(eta0)
  [delta_ksi_vec] -> cal lumped observation error agent 5/5(delta_ksi_vec)
  cal lumped observation error agent 4/2(eta_est_err_tilt_4) -> [eta_est_err_tilt_4]
  [eta_d_est_vec] -> cal lumped observation error agent 5/6(eta_d_est_vec)
  [ksi_est_err_tilt_1] -> "combine lumped follower observation error "/1(ksi_est_err_tilt_1)
  [delta_eta_vec] -> cal lumped observation error agent 5/8(delta_eta_vec)
  [delta_eta_vec] -> cal lumped observation error agent 2/8(delta_eta_vec)
  [ksi_est_err_tilt_3] -> "combine lumped follower observation error "/3(ksi_est_err_tilt_3)
  [ksi_est_err_tilt_2] -> "combine lumped follower observation error "/2(ksi_est_err_tilt_2)
  [delta_eta_vec] -> cal lumped observation error agent 3/8(delta_eta_vec)
  [delta_ksi_vec] -> cal lumped observation error agent 3/5(delta_ksi_vec)
  cal lumped observation error agent 2/1(ksi_est_err_tilt_2) -> [ksi_est_err_tilt_2]
  "combine lumped follower observation error "/1(ksi_est_err_tilt_vec) -> [ksi_est_err_tilt_vec]
  [ksi0] -> cal lumped observation error agent 2/4(ksi0)
  cal lumped observation error agent 2/2(eta_est_err_tilt_2) -> [eta_est_err_tilt_2]
  Constant242/1 -> cal lumped observation error agent 5/2(w0)
  [eta_est_err_tilt_4] -> "combine lumped follower observation error "/9(eta_est_err_tilt_4)
  [delta_eta_vec] -> cal lumped observation error agent 1/8(delta_eta_vec)
  [eta_d_est_vec] -> cal lumped observation error agent 1/6(eta_d_est_vec)
  Constant228/1 -> cal lumped observation error agent 2/2(w0)
  Constant233/1 -> cal lumped observation error agent 3/2(w0)
  Constant223/1 -> cal lumped observation error agent 1/1(wij)
  [ksi_d_est_vec] -> cal lumped observation error agent 2/3(ksi_d_est_vec)
  Constant237/1 -> cal lumped observation error agent 4/2(w0)
  [ksi_d_est_vec] -> cal lumped observation error agent 4/3(ksi_d_est_vec)
  [ksi_d_est_vec] -> cal lumped observation error agent 1/3(ksi_d_est_vec)
  [eta0] -> cal lumped observation error agent 3/7(eta0)
  [eta0] -> cal lumped observation error agent 2/7(eta0)
  [ksi_d_est_vec] -> cal lumped observation error agent 3/3(ksi_d_est_vec)
  cal lumped observation error agent 3/2(eta_est_err_tilt_3) -> [eta_est_err_tilt_3]
  [eta_est_err_tilt_1] -> "combine lumped follower observation error "/6(eta_est_err_tilt_1)
  cal lumped observation error agent 4/1(ksi_est_err_tilt_4) -> [ksi_est_err_tilt_4]
  cal lumped observation error agent 1/2(eta_est_err_tilt_1) -> [eta_est_err_tilt_1]
  [eta_d_est_vec] -> cal lumped observation error agent 3/6(eta_d_est_vec)
  Constant240/1 -> cal lumped observation error agent 5/1(wij)
  [ksi0] -> cal lumped observation error agent 5/4(ksi0)
  [eta_est_err_tilt_5] -> "combine lumped follower observation error "/10(eta_est_err_tilt_5)
  [eta_est_err_tilt_2] -> "combine lumped follower observation error "/7(eta_est_err_tilt_2)
  [eta0] -> cal lumped observation error agent 4/7(eta0)
  cal lumped observation error agent 1/1(ksi_est_err_tilt_1) -> [ksi_est_err_tilt_1]
  [eta0] -> cal lumped observation error agent 1/7(eta0)
  [theta_sigma_bar_v_tilt_2_vec] -> cal sigma_bar_v_hat agent 5/4(theta_sigma_bar_v_tilt_2_vec)
  [dp_hat_5] -> combine dp_hat/5(dp_hat_5)
  Constant113/1 -> cal theta_sigma_bar_v_tilt agent 4/1(alfa_theta)
  Constant119/1 -> Mux28/3
  [sigma_bar_v_vec] -> cal differentiator d_sigma_bar_v_hat agent 2/1(x)
  trans to column28/1(y) -> [sigma_bar_v_tilt_squ_2_5], Display58/1
  Demux12/2 -> d2_sigma_bar_v_est_1/2
  [d_sigma_bar_v_vec] -> cal dp_hat agent 5/2(d_sigma_bar_v_vec)
  [sigma_bar_v_tilt_squ_1_4] -> cal theta_sigma_bar_v_tilt agent 4/2(sigma_bar_v_tilt_squ_1_4)
  Demux4/3 -> d2_sigma_bar_v_est_3/3
  cal sigma_bar_v_hat agent 5/1(d_sigma_bar_v_hat_5) -> sigma_bar_v_hat Integrator 5/1
  cal dp_hat agent 1/1(dp_hat_1) -> [dp_hat_1]
  sigma_v Integrator 5/1 -> [sigma_v_5]
  cal theta_sigma_bar_v_tilt agent 1/2(theta_sigma_bar_v_tilt_2_1) -> [theta_sigma_bar_v_tilt_2_1]
  [sigma_bar_v_hat_vec] -> cal dp_hat agent 3/3(sigma_bar_v_hat_vec)
  cal theta_sigma_bar_v_tilt agent 1/1(theta_sigma_bar_v_tilt_1_1) -> [theta_sigma_bar_v_tilt_1_1]
  [theta_sigma_bar_v_tilt_2_vec] -> cal sigma_bar_v_hat agent 4/4(theta_sigma_bar_v_tilt_2_vec)
  [theta_sigma_bar_v_tilt_2_vec] -> cal sigma_bar_v_hat agent 3/4(theta_sigma_bar_v_tilt_2_vec)
  cal abs 30/1(y) -> Mux27/1
  [ui] -> cal virtual control sigma_v agent 1/3(ui_vec)
  Constant108/1 -> cal theta_sigma_bar_v_tilt agent 3/1(alfa_theta)
  choose ksi_est_err 27/1(y) -> cal abs 27/1(x)
  cal theta_sigma_bar_v_tilt agent 2/2(theta_sigma_bar_v_tilt_2_2) -> [theta_sigma_bar_v_tilt_2_2]
  Demux10/2 -> d_sigma_bar_v_est_5/2
  Mux19/1 -> Interpreted MATLAB Function20/1
  [dp_hat_3] -> combine dp_hat/3(dp_hat_3)
  Demux7/1 -> d_sigma_bar_v_est_4/1
  [sigma_bar_v_hat_vec] -> cal dp_hat agent 2/3(sigma_bar_v_hat_vec)
  sigma_bar_v_hat Integrator 4/1 -> [sigma_bar_v_hat_4]
  Constant109/1 -> Mux24/3
  [sigma_bar_v_hat_vec] -> cal dp_hat agent 1/3(sigma_bar_v_hat_vec)
  Interpreted MATLAB Function21/1 -> trans to column21/1(x)
  Demux10/1 -> d_sigma_bar_v_est_5/1
  cal sigma_bar_v_hat agent 3/1(d_sigma_bar_v_hat_3) -> sigma_bar_v_hat Integrator 3/1
  [sigma_bar_v_hat_3] -> combine sigma_bar_v_hat/3(sigma_bar_v_hat_3)
  [sigma_bar_v_vec] -> cal combine sigma_bar_v_tilt/1(sigma_bar_v_vec)
  Constant139/1 -> cal sigma_bar_v_hat agent 4/2(c2v)
  sigma_bar_v_hat Integrator 3/1 -> [sigma_bar_v_hat_3]
  [sigma_bar_v_hat_2] -> combine sigma_bar_v_hat/2(sigma_bar_v_hat_2)
  [theta_sigma_bar_v_tilt_1_vec] -> cal sigma_bar_v_hat agent 5/3(theta_sigma_bar_v_tilt_1_vec)
  [theta_sigma_bar_v_tilt_1_vec] -> cal sigma_bar_v_hat agent 4/3(theta_sigma_bar_v_tilt_1_vec)
  [d_sigma_bar_v_vec] -> cal sigma_bar_v_hat agent 3/5(d_sigma_bar_v_vec)
  Constant124/1 -> cal sigma_bar_v_hat agent 2/1(c1v)
  Constant125/1 -> cal sigma_bar_v_hat agent 2/2(c2v)
  Constant127/1 -> cal sigma_bar_v_hat agent 3/2(c2v)
  [theta_sigma_bar_v_tilt_2_vec] -> cal sigma_bar_v_hat agent 2/4(theta_sigma_bar_v_tilt_2_vec)
  [d_sigma_bar_v_vec] -> cal sigma_bar_v_hat agent 2/5(d_sigma_bar_v_vec)
  [theta_sigma_bar_v_tilt_1_vec] -> cal sigma_bar_v_hat agent 2/3(theta_sigma_bar_v_tilt_1_vec)
  [theta_sigma_bar_v_tilt_2_3] -> combine theta_sigma_bar_v_tilt/8(theta_sigma_bar_v_tilt_2_3)
  [theta_sigma_bar_v_tilt_1_3] -> combine theta_sigma_bar_v_tilt/3(theta_sigma_bar_v_tilt_1_3)
  Constant122/1 -> cal sigma_bar_v_hat agent 1/1(c1v)
  [d_sigma_bar_v_vec] -> cal sigma_bar_v_hat agent 1/5(d_sigma_bar_v_vec)
  [theta_sigma_bar_v_tilt_1_1] -> combine theta_sigma_bar_v_tilt/1(theta_sigma_bar_v_tilt_1_1)
  [theta_sigma_bar_v_tilt_1_5] -> combine theta_sigma_bar_v_tilt/5(theta_sigma_bar_v_tilt_1_5)
  [d_sigma_bar_v_est_5] -> combine d_sigma_bar_v_est/5(d_sigma_bar_v_est_5)
  combine theta_sigma_bar_v_tilt/2(theta_sigma_bar_v_tilt_2_vec) -> [theta_sigma_bar_v_tilt_2_vec]
  [theta_sigma_bar_v_tilt_2_1] -> combine theta_sigma_bar_v_tilt/6(theta_sigma_bar_v_tilt_2_1)
  Constant92/1 -> cal virtual control sigma_v agent 1/1(c3v)
  trans to column29/1(y) -> [sigma_bar_v_tilt_squ_1_5], Display59/1
  [theta_sigma_bar_v_tilt_1_2] -> combine theta_sigma_bar_v_tilt/2(theta_sigma_bar_v_tilt_1_2)
  [theta_sigma_bar_v_tilt_2_5] -> combine theta_sigma_bar_v_tilt/10(theta_sigma_bar_v_tilt_2_5)
  [theta_sigma_bar_v_tilt_2_2] -> combine theta_sigma_bar_v_tilt/7(theta_sigma_bar_v_tilt_2_2)
  [theta_sigma_bar_v_tilt_1_4] -> combine theta_sigma_bar_v_tilt/4(theta_sigma_bar_v_tilt_1_4)
  [sigma_bar_v_tilt_vec] -> choose ksi_est_err 30/1(x)
  [Ri] -> cal virtual control sigma_v agent 1/2(Ri)
  [sigma_bar_v_tilt_vec] -> cal theta_sigma_bar_v_tilt agent 5/4(sigma_bar_v_tilt_vec)
  Constant118/1 -> cal theta_sigma_bar_v_tilt agent 5/1(alfa_theta)
  [sigma_bar_v_tilt_vec] -> cal theta_sigma_bar_v_tilt agent 2/4(sigma_bar_v_tilt_vec)
  Interpreted MATLAB Function29/1 -> trans to column29/1(x)
  [sigma_bar_v_tilt_vec] -> choose ksi_est_err 29/1(x)
  [sigma_bar_v_vec] -> cal virtual control sigma_v agent 5/4(sigma_bar_v_vec)
  [d_sigma_bar_v_vec] -> cal dp_hat agent 4/2(d_sigma_bar_v_vec)
  [sigma_bar_v_tilt_squ_2_4] -> cal theta_sigma_bar_v_tilt agent 4/3(sigma_bar_v_tilt_squ_2_4)
  cal theta_sigma_bar_v_tilt agent 4/1(theta_sigma_bar_v_tilt_1_4) -> [theta_sigma_bar_v_tilt_1_4]
  Interpreted MATLAB Function28/1 -> trans to column28/1(x)
  [sigma_bar_v_tilt_vec] -> choose ksi_est_err 28/1(x)
  [sigma_bar_v_tilt_vec] -> cal theta_sigma_bar_v_tilt agent 4/4(sigma_bar_v_tilt_vec)
  [sigma_bar_v_tilt_vec] -> choose ksi_est_err 22/1(x)
  trans to column24/1(y) -> [sigma_bar_v_tilt_squ_2_3], Display54/1
  trans to column27/1(y) -> [sigma_bar_v_tilt_squ_1_4], Display57/1
  Mux26/1 -> Interpreted MATLAB Function27/1
  Constant116/1 -> Mux25/3
  [sigma_bar_v_tilt_vec] -> cal theta_sigma_bar_v_tilt agent 3/4(sigma_bar_v_tilt_vec)
  Demux12/3 -> d2_sigma_bar_v_est_1/3
  [d_sigma_bar_v_vec] -> cal sigma_bar_v_hat agent 4/5(d_sigma_bar_v_vec)
  [ui] -> cal virtual control sigma_v agent 2/3(ui_vec)
  trans to column23/1(y) -> [sigma_bar_v_tilt_squ_1_2], Display53/1
  cal abs 25/1(y) -> Mux24/1
  [sigma_bar_v_tilt_squ_2_3] -> cal theta_sigma_bar_v_tilt agent 3/3(sigma_bar_v_tilt_squ_2_3)
  Constant110/1 -> Mux23/2
  cal theta_sigma_bar_v_tilt agent 3/1(theta_sigma_bar_v_tilt_1_3) -> [theta_sigma_bar_v_tilt_1_3]
  Mux24/1 -> Interpreted MATLAB Function25/1
  Constant107/1 -> Mux24/2
  choose ksi_est_err 24/1(y) -> cal abs 24/1(x)
  [sigma_bar_v_tilt_vec] -> choose ksi_est_err 23/1(x)
  Constant105/1 -> Mux21/2
  Interpreted MATLAB Function22/1 -> trans to column22/1(x)
  [sigma_bar_v_tilt_vec] -> cal theta_sigma_bar_v_tilt agent 1/4(sigma_bar_v_tilt_vec)
  Mux20/1 -> Interpreted MATLAB Function21/1
  [sigma_bar_v_tilt_squ_1_1] -> cal theta_sigma_bar_v_tilt agent 1/2(sigma_bar_v_tilt_squ_1_1)
  Constant103/1 -> cal theta_sigma_bar_v_tilt agent 2/1(alfa_theta)
  Interpreted MATLAB Function23/1 -> trans to column23/1(x)
  Constant101/1 -> cal theta_sigma_bar_v_tilt agent 1/1(alfa_theta)
  [sigma_bar_v_tilt_squ_2_1] -> cal theta_sigma_bar_v_tilt agent 1/3(sigma_bar_v_tilt_squ_2_1)
  choose ksi_est_err 22/1(y) -> cal abs 22/1(x)
  cal abs 21/1(y) -> Mux20/1
  Constant99/1 -> Mux19/3
  Constant98/1 -> Mux19/2
  Interpreted MATLAB Function20/1 -> trans to column20/1(x)
  Constant97/1 -> Mux20/3
  Constant123/1 -> cal sigma_bar_v_hat agent 1/2(c2v)
  choose ksi_est_err 21/1(y) -> cal abs 21/1(x)
  [sigma_bar_v_tilt_vec] -> choose ksi_est_err 21/1(x)
  [theta_sigma_bar_v_tilt_2_4] -> combine theta_sigma_bar_v_tilt/9(theta_sigma_bar_v_tilt_2_4)
  [d_sigma_bar_v_est_3] -> combine d_sigma_bar_v_est/3(d_sigma_bar_v_est_3)
  sigma_bar_v_hat Integrator 5/1 -> [sigma_bar_v_hat_5]
  [d_sigma_bar_v_est_4] -> combine d_sigma_bar_v_est/4(d_sigma_bar_v_est_4)
  combine d_sigma_bar_v_est/1(d_sigma_bar_v_vec) -> [d_sigma_bar_v_vec]
  Demux10/3 -> d_sigma_bar_v_est_5/3
  [sigma_bar_v_hat_vec] -> cal combine sigma_bar_v_tilt/2(sigma_bar_v_hat_vec)
  Demux9/1 -> d2_sigma_bar_v_est_5/1
  [ui] -> cal virtual control sigma_v agent 3/3(ui_vec)
  [d_sigma_bar_v_est_2] -> combine d_sigma_bar_v_est/2(d_sigma_bar_v_est_2)
  cal theta_sigma_bar_v_tilt agent 4/2(theta_sigma_bar_v_tilt_2_4) -> [theta_sigma_bar_v_tilt_2_4]
  cal abs 29/1(y) -> Mux28/1
  cal differentiator d_sigma_bar_v_hat agent 5/3(Out3) -> Demux9/1, [d2_sigma_bar_v_est_5], Display49/1
  [sigma_bar_v_vec] -> cal differentiator d_sigma_bar_v_hat agent 5/1(x)
  Demux9/2 -> d2_sigma_bar_v_est_5/2
  Demux6/2 -> d2_sigma_bar_v_est_4/2
  cal differentiator d_sigma_bar_v_hat agent 3/1(Out1) -> Display41/1, [sigma_bar_v_est_3]
  Demux6/1 -> d2_sigma_bar_v_est_4/1
  cal differentiator d_sigma_bar_v_hat agent 4/3(Out3) -> Demux6/1, [d2_sigma_bar_v_est_4], Display46/1
  [sigma_bar_v_hat_4] -> combine sigma_bar_v_hat/4(sigma_bar_v_hat_4)
  cal differentiator d_sigma_bar_v_hat agent 3/2(Out2) -> Demux5/1, [d_sigma_bar_v_est_3], Display42/1
  [sigma_bar_v_vec] -> cal differentiator d_sigma_bar_v_hat agent 4/1(x)
  cal differentiator d_sigma_bar_v_hat agent 1/2(Out2) -> Demux8/1, [d_sigma_bar_v_est_1], Display36/1
  Constant102/1 -> Mux22/2
  cal sigma_bar_v_hat agent 4/1(d_sigma_bar_v_hat_4) -> sigma_bar_v_hat Integrator 4/1
  Demux5/3 -> d_sigma_bar_v_est_3/3
  cal differentiator d_sigma_bar_v_hat agent 2/1(Out1) -> Display38/1, [sigma_bar_v_est_2]
  Mux21/1 -> Interpreted MATLAB Function22/1
  [sigma_bar_v_vec] -> cal differentiator d_sigma_bar_v_hat agent 1/1(x)
  [sigma_bar_v_tilt_vec] -> choose ksi_est_err 24/1(x)
  Demux2/3 -> d2_sigma_bar_v_est_2/3
  cal combine sigma_bar_v/1(sigma_bar_v_vec) -> [sigma_bar_v_vec]
  [sigma_v_1] -> combine sigma_v/1(sigma_v_1)
  Mux22/1 -> Interpreted MATLAB Function23/1
  Demux8/1 -> d_sigma_bar_v_est_1/1
  Demux12/1 -> d2_sigma_bar_v_est_1/1
  [sigma_v_5] -> combine sigma_v/5(sigma_v_5)
  Demux8/3 -> d_sigma_bar_v_est_1/3
  cal differentiator d_sigma_bar_v_hat agent 1/1(Out1) -> Display35/1, [sigma_bar_v_est_1]
  [sigma_bar_v_tilt_squ_1_2] -> cal theta_sigma_bar_v_tilt agent 2/2(sigma_bar_v_tilt_squ_1_2)
  combine dp_hat/1(dp_hat_vec) -> [dp_hat_vec]
  [dp_hat_4] -> combine dp_hat/4(dp_hat_4)
  [sigma_bar_v_hat_vec] -> cal dp_hat agent 5/3(sigma_bar_v_hat_vec)
  choose ksi_est_err 25/1(y) -> cal abs 25/1(x)
  Constant145/1 -> cal dp_hat agent 4/1(c3v)
  cal dp_hat agent 4/1(dp_hat_4) -> [dp_hat_4]
  Demux8/2 -> d_sigma_bar_v_est_1/2
  [d_sigma_bar_v_vec] -> cal dp_hat agent 2/2(d_sigma_bar_v_vec)
  cal dp_hat agent 3/1(dp_hat_3) -> [dp_hat_3]
  [d_sigma_bar_v_vec] -> cal dp_hat agent 1/2(d_sigma_bar_v_vec)
  trans to column21/1(y) -> [sigma_bar_v_tilt_squ_1_1], Display51/1
  Demux3/3 -> d_sigma_bar_v_est_2/3
  Mux25/1 -> Interpreted MATLAB Function26/1
  cal dp_hat agent 2/1(dp_hat_2) -> [dp_hat_2]
  Constant104/1 -> Mux22/3
  [Ri] -> cal virtual control sigma_v agent 5/2(Ri)
  Constant143/1 -> cal dp_hat agent 2/1(c3v)
  Constant144/1 -> cal dp_hat agent 3/1(c3v)
  Constant142/1 -> cal dp_hat agent 1/1(c3v)
  Constant126/1 -> cal sigma_bar_v_hat agent 3/1(c1v)
  Constant140/1 -> cal sigma_bar_v_hat agent 5/1(c1v)
  [dp_hat_2] -> combine dp_hat/2(dp_hat_2)
  cal abs 28/1(y) -> Mux25/1
  cal abs 22/1(y) -> Mux19/1
  sigma_bar_v_hat Integrator 2/1 -> [sigma_bar_v_hat_2]
  Mux27/1 -> Interpreted MATLAB Function28/1
  Constant106/1 -> Mux21/3
  Demux3/2 -> d_sigma_bar_v_est_2/2
  [Ri] -> cal virtual control sigma_v agent 3/2(Ri)
  cal theta_sigma_bar_v_tilt agent 5/1(theta_sigma_bar_v_tilt_1_5) -> [theta_sigma_bar_v_tilt_1_5]
  Constant111/1 -> Mux23/3
  Demux5/1 -> d_sigma_bar_v_est_3/1
  cal sigma_bar_v_hat agent 1/1(d_sigma_bar_v_hat_1) -> sigma_bar_v_hat Integrator 1/1
  cal differentiator d_sigma_bar_v_hat agent 5/2(Out2) -> Demux10/1, [d_sigma_bar_v_est_5], Display48/1
  [Ri] -> cal virtual control sigma_v agent 4/2(Ri)
  [sigma_bar_v_hat_vec] -> cal dp_hat agent 4/3(sigma_bar_v_hat_vec)
  cal abs 26/1(y) -> Mux23/1
  Demux5/2 -> d_sigma_bar_v_est_3/2
  [dp_hat_1] -> combine dp_hat/1(dp_hat_1)
  cal abs 27/1(y) -> Mux26/1
  Demux3/1 -> d_sigma_bar_v_est_2/1
  Constant100/1 -> Mux20/2
  [sigma_bar_v_tilt_vec] -> choose ksi_est_err 26/1(x)
  Constant114/1 -> Mux26/3
  Interpreted MATLAB Function25/1 -> trans to column25/1(x)
  Demux6/3 -> d2_sigma_bar_v_est_4/3
  cal differentiator d_sigma_bar_v_hat agent 3/3(Out3) -> Demux4/1, [d2_sigma_bar_v_est_3], Display43/1
  Constant120/1 -> Mux27/2
  choose ksi_est_err 26/1(y) -> cal abs 26/1(x)
  Constant115/1 -> Mux25/2
  [sigma_bar_v_tilt_squ_2_5] -> cal theta_sigma_bar_v_tilt agent 5/3(sigma_bar_v_tilt_squ_2_5)
  Demux2/2 -> d2_sigma_bar_v_est_2/2
  Constant128/1 -> cal sigma_bar_v_hat agent 4/1(c1v)
  choose ksi_est_err 28/1(y) -> cal abs 28/1(x)
  Demux2/1 -> d2_sigma_bar_v_est_2/1
  [theta_sigma_bar_v_tilt_1_vec] -> cal sigma_bar_v_hat agent 1/3(theta_sigma_bar_v_tilt_1_vec)
  Demux9/3 -> d2_sigma_bar_v_est_5/3
  [sigma_v_vec] -> cal combine sigma_bar_v/2(sigma_v_vec)
  [sigma_v_2] -> combine sigma_v/2(sigma_v_2)
  combine theta_sigma_bar_v_tilt/1(theta_sigma_bar_v_tilt_1_vec) -> [theta_sigma_bar_v_tilt_1_vec]
  Interpreted MATLAB Function26/1 -> trans to column26/1(x)
  Demux4/1 -> d2_sigma_bar_v_est_3/1
  [sigma_bar_v_tilt_vec] -> choose ksi_est_err 27/1(x)
  [d_sigma_bar_v_vec] -> cal sigma_bar_v_hat agent 5/5(d_sigma_bar_v_vec)
  cal differentiator d_sigma_bar_v_hat agent 2/2(Out2) -> Demux3/1, [d_sigma_bar_v_est_2], Display39/1
  Constant93/1 -> cal virtual control sigma_v agent 2/1(c3v)
  trans to column20/1(y) -> [sigma_bar_v_tilt_squ_2_1], Display50/1
  cal virtual control sigma_v agent 5/1(d_sigma_v_5) -> sigma_v Integrator 5/1
  [d_sigma_bar_v_vec] -> cal dp_hat agent 3/2(d_sigma_bar_v_vec)
  Constant112/1 -> Mux26/2
  Mux28/1 -> Interpreted MATLAB Function29/1
  choose ksi_est_err 30/1(y) -> cal abs 30/1(x)
  [eta_i_vec] -> cal combine sigma_bar_v/1(eta_i_vec)
  Constant121/1 -> Mux27/3
  [sigma_bar_v_hat_1] -> combine sigma_bar_v_hat/1(sigma_bar_v_hat_1)
  cal differentiator d_sigma_bar_v_hat agent 5/1(Out1) -> Display47/1, [sigma_bar_v_est_5]
  cal theta_sigma_bar_v_tilt agent 3/2(theta_sigma_bar_v_tilt_2_3) -> [theta_sigma_bar_v_tilt_2_3]
  Constant146/1 -> cal dp_hat agent 5/1(c3v)
  trans to column26/1(y) -> [sigma_bar_v_tilt_squ_2_4], Display56/1
  [d_sigma_bar_v_est_1] -> combine d_sigma_bar_v_est/1(d_sigma_bar_v_est_1)
  Constant141/1 -> cal sigma_bar_v_hat agent 5/2(c2v)
  cal differentiator d_sigma_bar_v_hat agent 2/3(Out3) -> Demux2/1, [d2_sigma_bar_v_est_2], Display40/1
  [sigma_bar_v_tilt_vec] -> choose ksi_est_err 25/1(x)
  [sigma_bar_v_tilt_squ_2_2] -> cal theta_sigma_bar_v_tilt agent 2/3(sigma_bar_v_tilt_squ_2_2)
  Constant95/1 -> cal virtual control sigma_v agent 4/1(c3v)
  cal combine sigma_bar_v_tilt/1(sigma_bar_v_tilt_vec) -> [sigma_bar_v_tilt_vec]
  cal virtual control sigma_v agent 3/1(d_sigma_v_3) -> sigma_v Integrator 3/1
  cal differentiator d_sigma_bar_v_hat agent 4/1(Out1) -> Display44/1, [sigma_bar_v_est_4]
  cal theta_sigma_bar_v_tilt agent 5/2(theta_sigma_bar_v_tilt_2_5) -> [theta_sigma_bar_v_tilt_2_5]
  [theta_sigma_bar_v_tilt_2_vec] -> cal sigma_bar_v_hat agent 1/4(theta_sigma_bar_v_tilt_2_vec)
  [sigma_v_4] -> combine sigma_v/4(sigma_v_4)
  trans to column25/1(y) -> [sigma_bar_v_tilt_squ_1_3], Display55/1
  cal differentiator d_sigma_bar_v_hat agent 1/3(Out3) -> Demux12/1, [d2_sigma_bar_v_est_1], Display37/1
  [theta_sigma_bar_v_tilt_1_vec] -> cal sigma_bar_v_hat agent 3/3(theta_sigma_bar_v_tilt_1_vec)
  trans to column22/1(y) -> [sigma_bar_v_tilt_squ_2_2], Display52/1
  [sigma_bar_v_tilt_squ_1_3] -> cal theta_sigma_bar_v_tilt agent 3/2(sigma_bar_v_tilt_squ_1_3)
  cal abs 23/1(y) -> Mux22/1
  Demux4/2 -> d2_sigma_bar_v_est_3/2
  cal dp_hat agent 5/1(dp_hat_5) -> [dp_hat_5]
  [sigma_bar_v_vec] -> cal differentiator d_sigma_bar_v_hat agent 3/1(x)
  Interpreted MATLAB Function24/1 -> trans to column24/1(x)
  cal virtual control sigma_v agent 4/1(d_sigma_v_4) -> sigma_v Integrator 4/1
  Mux23/1 -> Interpreted MATLAB Function24/1
  [sigma_bar_v_vec] -> cal virtual control sigma_v agent 3/4(sigma_bar_v_vec)
  [sigma_bar_v_vec] -> cal virtual control sigma_v agent 4/4(sigma_bar_v_vec)
  Constant94/1 -> cal virtual control sigma_v agent 3/1(c3v)
  Demux7/2 -> d_sigma_bar_v_est_4/2
  sigma_bar_v_hat Integrator 1/1 -> [sigma_bar_v_hat_1]
  [ui] -> cal virtual control sigma_v agent 4/3(ui_vec)
  cal abs 24/1(y) -> Mux21/1
  sigma_v Integrator 4/1 -> [sigma_v_4]
  cal theta_sigma_bar_v_tilt agent 2/1(theta_sigma_bar_v_tilt_1_2) -> [theta_sigma_bar_v_tilt_1_2]
  sigma_v Integrator 3/1 -> [sigma_v_3]
  cal sigma_bar_v_hat agent 2/1(d_sigma_bar_v_hat_2) -> sigma_bar_v_hat Integrator 2/1
  [Ri] -> cal virtual control sigma_v agent 2/2(Ri)
  Interpreted MATLAB Function27/1 -> trans to column27/1(x)
  [sigma_bar_v_hat_5] -> combine sigma_bar_v_hat/5(sigma_bar_v_hat_5)
  [sigma_bar_v_vec] -> cal virtual control sigma_v agent 2/4(sigma_bar_v_vec)
  Constant117/1 -> Mux28/2
  Demux7/3 -> d_sigma_bar_v_est_4/3
  [sigma_bar_v_vec] -> cal virtual control sigma_v agent 1/4(sigma_bar_v_vec)
  [sigma_bar_v_tilt_squ_1_5] -> cal theta_sigma_bar_v_tilt agent 5/2(sigma_bar_v_tilt_squ_1_5)
  Constant96/1 -> cal virtual control sigma_v agent 5/1(c3v)
  sigma_v Integrator 2/1 -> [sigma_v_2]
  combine sigma_v/1(sigma_v_vec) -> [sigma_v_vec]
  cal virtual control sigma_v agent 1/1(d_sigma_v_1) -> sigma_v Integrator 1/1
  choose ksi_est_err 29/1(y) -> cal abs 29/1(x)
  cal virtual control sigma_v agent 2/1(d_sigma_v_2) -> sigma_v Integrator 2/1
  choose ksi_est_err 23/1(y) -> cal abs 23/1(x)
  [sigma_v_3] -> combine sigma_v/3(sigma_v_3)
  sigma_v Integrator 1/1 -> [sigma_v_1]
  cal differentiator d_sigma_bar_v_hat agent 4/2(Out2) -> Demux7/1, [d_sigma_bar_v_est_4], Display45/1
  [ui] -> cal virtual control sigma_v agent 5/3(ui_vec)
  combine sigma_bar_v_hat/1(sigma_bar_v_hat_vec) -> [sigma_bar_v_hat_vec]
  Demux31/2 -> ksi_track_err_5/2
  [dp_5] -> combine translational disturbance/5(dp_5)
  [ui] -> uav translational dynamics agent 3/2(ui)
  [dp_vec] -> uav translational dynamics agent 4/3(dp)
  [ui] -> uav translational dynamics agent 2/2(ui)
  [dp_vec] -> uav translational dynamics agent 5/3(dp)
  follower tracking error agent 2/2(eta_track_err_2) -> Display15/1, Demux26/1, [eta_track_err_2]
  [eta_track_err_1] -> combine follower eta ksi/6(eta_track_err_1)
  Demux26/2 -> eta_track_err_2/2
  generate translational disturbance agent 1/1(dp_1) -> [dp_1]
  Demux30/1 -> eta_track_err_4/1
  [eta_1] -> combine formation control input/1(eta_1)
  [eta_3] -> combine formation control input/3(eta_3)
  [ksi_1] -> combine formation control input/6(ksi_1)
  follower tracking error agent 4/2(eta_track_err_4) -> Display19/1, Demux30/1, [eta_track_err_4]
  [ksi0] -> follower tracking error agent 2/5(ksi0)
  uav translational dynamics agent 1/1(dvi) -> follower etai Integrator agent 1/1
  follower tracking error agent 3/2(eta_track_err_3) -> Display17/1, Demux28/1, [eta_track_err_3]
  [dp_vec] -> uav translational dynamics agent 1/3(dp)
  Demux27/2 -> ksi_track_err_3/2
  [dp_hat_vec] -> cal disturbance observation error dp_tilt/2(dp_hat_vec)
  Demux32/1 -> eta_track_err_5/1
  [eta_5] -> combine formation control input/5(eta_5)
  follower ksii Integrator agent 4/1 -> [ksi_4]
  [ksi0] -> follower tracking error agent 1/5(ksi0)
  [dp_3] -> combine translational disturbance/3(dp_3)
  [Ri] -> uav translational dynamics agent 1/1(Ri)
  [ksi0] -> follower tracking error agent 5/5(ksi0)
  Demux26/1 -> eta_track_err_2/1
  [ksi_i_vec] -> follower tracking error agent 5/3(ksi_i_vec)
  Demux31/3 -> ksi_track_err_5/3
  follower ksii Integrator agent 1/1 -> [ksi_1]
  Demux28/1 -> eta_track_err_3/1
  follower tracking error agent 2/1(ksi_track_err_2) -> Display14/1, Demux25/1, [ksi_track_err_2]
  cal disturbance observation error dp_tilt/1(dp_tilt_vec) -> [dp_tilt_vec]
  [eta_4] -> combine formation control input/4(eta_4)
  [dp_vec] -> cal disturbance observation error dp_tilt/1(dp_vec)
  uav translational dynamics agent 3/1(dvi) -> follower etai Integrator agent 3/1
  follower tracking error agent 1/1(ksi_track_err_1) -> Display12/1, Demux23/1, [ksi_track_err_1]
  [delta_ksi_vec] -> follower tracking error agent 1/1(delta_ksi_vec)
  follower etai Integrator agent 2/1 -> [eta_2], follower ksii Integrator agent 2/1
  [ksi_track_err_4] -> combine follower eta ksi/4(ksi_track_err_4)
  [dp_vec] -> uav translational dynamics agent 3/3(dp)
  generate translational disturbance agent 5/1(dp_5) -> [dp_5]
  [tsim] -> generate translational disturbance agent 5/4(t)
  [eta0] -> follower tracking error agent 4/6(eta0)
  [delta_eta_vec] -> follower tracking error agent 3/2(delta_eta_vec)
  Constant291/1 -> generate translational disturbance agent 3/1(dp_aa_t)
  Constant296/1 -> generate translational disturbance agent 5/2(dp_ff_t)
  Constant297/1 -> generate translational disturbance agent 5/1(dp_aa_t)
  Constant295/1 -> generate translational disturbance agent 5/3(dp_phi_t)
  Constant292/1 -> generate translational disturbance agent 4/3(dp_phi_t)
  Constant286/1 -> generate translational disturbance agent 2/3(dp_phi_t)
  Constant293/1 -> generate translational disturbance agent 4/2(dp_ff_t)
  [eta_2] -> combine formation control input/2(eta_2)
  Constant244/1 -> generate translational disturbance agent 1/2(dp_ff_t)
  Constant289/1 -> generate translational disturbance agent 3/3(dp_phi_t)
  [delta_ksi_vec] -> follower tracking error agent 5/1(delta_ksi_vec)
  [eta_track_err_5] -> combine follower eta ksi/10(eta_track_err_5)
  generate translational disturbance agent 4/1(dp_4) -> [dp_4]
  Constant294/1 -> generate translational disturbance agent 4/1(dp_aa_t)
  [eta_i_vec] -> follower tracking error agent 2/4(eta_i_vec)
  generate translational disturbance agent 3/1(dp_3) -> [dp_3]
  [eta_track_err_4] -> combine follower eta ksi/9(eta_track_err_4)
  [tsim] -> generate translational disturbance agent 4/4(t)
  generate translational disturbance agent 2/1(dp_2) -> [dp_2]
  Constant288/1 -> generate translational disturbance agent 2/1(dp_aa_t)
  [tsim] -> generate translational disturbance agent 2/4(t)
  Constant290/1 -> generate translational disturbance agent 3/2(dp_ff_t)
  Constant285/1 -> generate translational disturbance agent 1/1(dp_aa_t)
  Demux23/1 -> ksi_track_err_1/1
  [delta_eta_vec] -> follower tracking error agent 5/2(delta_eta_vec)
  Constant243/1 -> generate translational disturbance agent 1/3(dp_phi_t)
  [delta_ksi_vec] -> follower tracking error agent 3/1(delta_ksi_vec)
  [delta_ksi_vec] -> follower tracking error agent 4/1(delta_ksi_vec)
  follower etai Integrator agent 1/1 -> [eta_1], follower ksii Integrator agent 1/1
  [delta_ksi_vec] -> follower tracking error agent 2/1(delta_ksi_vec)
  [delta_eta_vec] -> follower tracking error agent 4/2(delta_eta_vec)
  Demux25/3 -> ksi_track_err_2/3
  [ksi_i_vec] -> follower tracking error agent 4/3(ksi_i_vec)
  [delta_eta_vec] -> follower tracking error agent 2/2(delta_eta_vec)
  follower ksii Integrator agent 5/1 -> [ksi_5]
  Demux25/2 -> ksi_track_err_2/2
  [dp_2] -> combine translational disturbance/2(dp_2)
  combine follower eta ksi/2(eta_track_err_vec) -> [eta_track_err_vec]
  Demux30/3 -> eta_track_err_4/3
  [ksi_4] -> combine formation control input/9(ksi_4)
  follower etai Integrator agent 3/1 -> [eta_3], follower ksii Integrator agent 3/1
  [dp_1] -> combine translational disturbance/1(dp_1)
  Demux27/3 -> ksi_track_err_3/3
  Demux30/2 -> eta_track_err_4/2
  [tsim] -> generate translational disturbance agent 1/4(t)
  Demux28/3 -> eta_track_err_3/3
  combine translational disturbance/1(dp_vec) -> [dp_vec]
  uav translational dynamics agent 4/1(dvi) -> follower etai Integrator agent 4/1
  [eta_i_vec] -> follower tracking error agent 5/4(eta_i_vec)
  [Ri] -> uav translational dynamics agent 4/1(Ri)
  [ui] -> uav translational dynamics agent 1/2(ui)
  Memory1/1 -> [eta_i_vec]
  combine formation control input/1(eta_i_vec) -> Memory1/1
  [ui] -> uav translational dynamics agent 4/2(ui)
  [Ri] -> uav translational dynamics agent 3/1(Ri)
  [Ri] -> uav translational dynamics agent 5/1(Ri)
  Memory2/1 -> [ksi_i_vec]
  [Ri] -> uav translational dynamics agent 2/1(Ri)
  Demux32/3 -> eta_track_err_5/3
  Demux27/1 -> ksi_track_err_3/1
  [tsim] -> generate translational disturbance agent 3/4(t)
  Demux31/1 -> ksi_track_err_5/1
  Demux25/1 -> ksi_track_err_2/1
  [ui] -> uav translational dynamics agent 5/2(ui)
  follower etai Integrator agent 5/1 -> [eta_5], follower ksii Integrator agent 5/1
  [eta_track_err_2] -> combine follower eta ksi/7(eta_track_err_2)
  [ksi_track_err_1] -> combine follower eta ksi/1(ksi_track_err_1)
  [ksi_track_err_5] -> combine follower eta ksi/5(ksi_track_err_5)
  [eta_track_err_3] -> combine follower eta ksi/8(eta_track_err_3)
  Demux28/2 -> eta_track_err_3/2
  [ksi_track_err_2] -> combine follower eta ksi/2(ksi_track_err_2)
  Constant287/1 -> generate translational disturbance agent 2/2(dp_ff_t)
  combine follower eta ksi/1(ksi_track_err_vec) -> [ksi_track_err_vec]
  [ksi_track_err_3] -> combine follower eta ksi/3(ksi_track_err_3)
  Demux29/1 -> ksi_track_err_4/1
  [ksi_3] -> combine formation control input/8(ksi_3)
  Demux29/2 -> ksi_track_err_4/2
  Demux24/1 -> eta_track_err_1/1
  [ksi_i_vec] -> follower tracking error agent 3/3(ksi_i_vec)
  Demux24/3 -> eta_track_err_1/3
  [ksi0] -> follower tracking error agent 4/5(ksi0)
  uav translational dynamics agent 5/1(dvi) -> follower etai Integrator agent 5/1
  follower tracking error agent 4/1(ksi_track_err_4) -> Display18/1, Demux29/1, [ksi_track_err_4]
  Demux29/3 -> ksi_track_err_4/3
  follower tracking error agent 5/1(ksi_track_err_5) -> Display20/1, Demux31/1, [ksi_track_err_5]
  [eta0] -> follower tracking error agent 3/6(eta0)
  Demux24/2 -> eta_track_err_1/2
  follower tracking error agent 3/1(ksi_track_err_3) -> Display16/1, Demux27/1, [ksi_track_err_3]
  uav translational dynamics agent 2/1(dvi) -> follower etai Integrator agent 2/1
  [ksi0] -> follower tracking error agent 3/5(ksi0)
  Demux26/3 -> eta_track_err_2/3
  [ksi_i_vec] -> follower tracking error agent 2/3(ksi_i_vec)
  [dp_vec] -> uav translational dynamics agent 2/3(dp)
  [eta_i_vec] -> follower tracking error agent 3/4(eta_i_vec)
  [eta_i_vec] -> follower tracking error agent 4/4(eta_i_vec)
  [ksi_i_vec] -> follower tracking error agent 1/3(ksi_i_vec)
  Demux32/2 -> eta_track_err_5/2
  follower tracking error agent 5/2(eta_track_err_5) -> Display21/1, Demux32/1, [eta_track_err_5]
  follower ksii Integrator agent 2/1 -> [ksi_2]
  [delta_eta_vec] -> follower tracking error agent 1/2(delta_eta_vec)
  follower tracking error agent 1/2(eta_track_err_1) -> Display13/1, Demux24/1, [eta_track_err_1]
  [dp_4] -> combine translational disturbance/4(dp_4)
  [eta0] -> follower tracking error agent 2/6(eta0)
  follower etai Integrator agent 4/1 -> [eta_4], follower ksii Integrator agent 4/1
  Demux23/3 -> ksi_track_err_1/3
  [ksi_5] -> combine formation control input/10(ksi_5)
  follower ksii Integrator agent 3/1 -> [ksi_3]
  Demux23/2 -> ksi_track_err_1/2
  [eta_i_vec] -> follower tracking error agent 1/4(eta_i_vec)
  [eta0] -> follower tracking error agent 5/6(eta0)
  [eta0] -> follower tracking error agent 1/6(eta0)
  combine formation control input/2(ksi_i_vec) -> Memory2/1
  [ksi_2] -> combine formation control input/7(ksi_2)
  [ksi0] -> cal position estimate error/2(ksi0)
  [eta_d_est_vec] -> cal velocity estimate error/1(eta_d_est_vec)
  [ksi_d_est_vec] -> cal position estimate error/1(ksi_d_est_vec)
  [eta0] -> cal velocity estimate error/2(eta0)
  cal velocity estimate error/1(eta_est_err) -> [eta_est_err]
  [delta_ksi_vec] -> cal position estimate error/3(delta_ksi_vec)
  cal position estimate error/1(ksi_est_err) -> [ksi_est_err]
  [delta_eta_vec] -> cal velocity estimate error/3(delta_eta_vec)
  set desire formation configuration/3(d_delta_eta_vec) -> [d_delta_eta_vec]
  [d_delta_eta_vec] -> cal ui agent 1/2(d_delta_eta_vec)
  [eps_p_hat_vec] -> cal ui agent 2/4(eps_p_hat_vec)
  [d_delta_eta_vec] -> cal ui agent 2/2(d_delta_eta_vec)
  [dp_hat_vec] -> cal ui agent 2/6(dp_hat_vec)
  Constant18/1 -> cal ui agent 2/1(c_psi_p)
  cal ui agent 2/1(ui_2) -> [ui_2]
  [err_Gi_form_vec] -> cal ui agent 2/3(err_Gi_form_vec)
  [err_lump_vec] -> cal ui agent 2/5(err_lump_vec)
  [err_Gi_form_vec] -> cal ui agent 3/3(err_Gi_form_vec)
  [dp_hat_vec] -> cal ui agent 3/6(dp_hat_vec)
  [d_delta_eta_vec] -> cal ui agent 3/2(d_delta_eta_vec)
  cal ui agent 3/1(ui_3) -> [ui_3]
  [eps_p_hat_vec] -> cal ui agent 3/4(eps_p_hat_vec)
  Constant19/1 -> cal ui agent 3/1(c_psi_p)
  [err_lump_vec] -> cal ui agent 3/5(err_lump_vec)
  Constant20/1 -> cal ui agent 4/1(c_psi_p)
  [err_lump_vec] -> cal ui agent 4/5(err_lump_vec)
  cal ui agent 4/1(ui_4) -> [ui_4]
  [d_delta_eta_vec] -> cal ui agent 4/2(d_delta_eta_vec)
  [dp_hat_vec] -> cal ui agent 4/6(dp_hat_vec)
  [err_Gi_form_vec] -> cal ui agent 4/3(err_Gi_form_vec)
  [eps_p_hat_vec] -> cal ui agent 4/4(eps_p_hat_vec)
  [eps_p_hat_vec] -> cal ui agent 5/4(eps_p_hat_vec)
  Constant21/1 -> cal ui agent 5/1(c_psi_p)
  [dp_hat_vec] -> cal ui agent 5/6(dp_hat_vec)
  [err_Gi_form_vec] -> cal ui agent 5/3(err_Gi_form_vec)
  cal ui agent 5/1(ui_5) -> [ui_5]
  [d_delta_eta_vec] -> cal ui agent 5/2(d_delta_eta_vec)
  [err_lump_vec] -> cal ui agent 5/5(err_lump_vec)
